simulink model "ForwardKinematic_YuMi"  (R2024a)
(part 14 of 23)

(4872700232219253*sin(q1L))/9007199254740992))/36893488147419103232 - (76229820211215127867025072518845*cos(q2L))/162259276829213363391578010288128 + sin(q2L)*((4872700232219253*cos(q1L))/9007199254740992 + (6283307137322267*sin(q1L))/9007199254740992)))/36893488147419103232))/36893488147419103232))/2451992865385422173373355243440494693789982595493763481600 + (27*cos(q5L)*(((7514214926474921*cos(q4L))/36893488147419103232 + (4503599440548691*sin(q4L))/4503599627370496)*((9007199067919185*cos(q3L)*((56594998190739085871744456992395*cos(q1L))/81129638414606681695789005144064 - (43889380989894851923989405068805*sin(q1L))/81129638414606681695789005144064 + 63594381400292563045725890951477/664613997892457936451903530140172288))/9007199254740992 + (7514214926474921*cos(q3L)*((7514214926474921*cos(q2L)*((6283307137322267*cos(q1L))/9007199254740992 - (4872700232219253*sin(q1L))/9007199254740992))/36893488147419103232 - (76229820211215127867025072518845*cos(q2L))/162259276829213363391578010288128 + sin(q2L)*((4872700232219253*cos(q1L))/9007199254740992 + (6283307137322267*sin(q1L))/9007199254740992)))/36893488147419103232 - sin(q3L)*((76229820211215127867025072518845*sin(q2L))/162259276829213363391578010288128 + cos(q2L)*((4872700232219253*cos(q1L))/9007199254740992 + (6283307137322267*sin(q1L))/9007199254740992) - (7514214926474921*sin(q2L)*((6283307137322267*cos(q1L))/9007199254740992 - (4872700232219253*sin(q1L))/9007199254740992))/36893488147419103232)) - (7514214926474921*sin(q4L)*((9007199067919185*sin(q3L)*((56594998190739085871744456992395*cos(q1L))/81129638414606681695789005144064 - (43889380989894851923989405068805*sin(q1L))/81129638414606681695789005144064 + 63594381400292563045725890951477/664613997892457936451903530140172288))/9007199254740992 + cos(q3L)*((76229820211215127867025072518845*sin(q2L))/162259276829213363391578010288128 + cos(q2L)*((4872700232219253*cos(q1L))/9007199254740992 + (6283307137322267*sin(q1L))/9007199254740992) - (7514214926474921*sin(q2L)*((6283307137322267*cos(q1L))/9007199254740992 - (4872700232219253*sin(q1L))/9007199254740992))/36893488147419103232) + (7514214926474921*sin(q3L)*((7514214926474921*cos(q2L)*((6283307137322267*cos(q1L))/9007199254740992 - (4872700232219253*sin(q1L))/9007199254740992))/36893488147419103232 - (76229820211215127867025072518845*cos(q2L))/162259276829213363391578010288128 + sin(q2L)*((4872700232219253*cos(q1L))/9007199254740992 + (6283307137322267*sin(q1L))/9007199254740992)))/36893488147419103232))/36893488147419103232))/1000 - (202883803014822867*sin(q5L)*(((4503599440548691*cos(q4L))/4503599627370496 - (7514214926474921*sin(q4L))/36893488147419103232)*((9007199067919185*cos(q3L)*((56594998190739085871744456992395*cos(q1L))/81129638414606681695789005144064 - (43889380989894851923989405068805*sin(q1L))/81129638414606681695789005144064 + 63594381400292563045725890951477/664613997892457936451903530140172288))/9007199254740992 + (7514214926474921*cos(q3L)*((7514214926474921*cos(q2L)*((6283307137322267*cos(q1L))/9007199254740992 - (4872700232219253*sin(q1L))/9007199254740992))/36893488147419103232 - (76229820211215127867025072518845*cos(q2L))/162259276829213363391578010288128 + sin(q2L)*((4872700232219253*cos(q1L))/9007199254740992 + (6283307137322267*sin(q1L))/9007199254740992)))/36893488147419103232 - sin(q3L)*((76229820211215127867025072518845*sin(q2L))/162259276829213363391578010288128 + cos(q2L)*((4872700232219253*cos(q1L))/9007199254740992 + (6283307137322267*sin(q1L))/9007199254740992) - (7514214926474921*sin(q2L)*((6283307137322267*cos(q1L))/9007199254740992 - (4872700232219253*sin(q1L))/9007199254740992))/36893488147419103232)) - (7514214926474921*cos(q4L)*((9007199067919185*sin(q3L)*((56594998190739085871744456992395*cos(q1L))/81129638414606681695789005144064 - (43889380989894851923989405068805*sin(q1L))/81129638414606681695789005144064 + 63594381400292563045725890951477/664613997892457936451903530140172288))/9007199254740992 + cos(q3L)*((76229820211215127867025072518845*sin(q2L))/162259276829213363391578010288128 + cos(q2L)*((4872700232219253*cos(q1L))/9007199254740992 + (6283307137322267*sin(q1L))/9007199254740992) - (7514214926474921*sin(q2L)*((6283307137322267*cos(q1L))/9007199254740992 - (4872700232219253*sin(q1L))/9007199254740992))/36893488147419103232) + (7514214926474921*sin(q3L)*((7514214926474921*cos(q2L)*((6283307137322267*cos(q1L))/9007199254740992 - (4872700232219253*sin(q1L))/9007199254740992))/36893488147419103232 - (76229820211215127867025072518845*cos(q2L))/162259276829213363391578010288128 + sin(q2L)*((4872700232219253*cos(q1L))/9007199254740992 + (6283307137322267*sin(q1L))/9007199254740992)))/36893488147419103232))/36893488147419103232))/36893488147419103232000 + (94754841554645069948206780163139*sin(q5L)*(((7514214926474921*cos(q4L))/36893488147419103232 + (4503599440548691*sin(q4L))/4503599627370496)*((9007199067919185*cos(q3L)*((56594998190739085871744456992395*cos(q1L))/81129638414606681695789005144064 - (43889380989894851923989405068805*sin(q1L))/81129638414606681695789005144064 + 63594381400292563045725890951477/664613997892457936451903530140172288))/9007199254740992 + (7514214926474921*cos(q3L)*((7514214926474921*cos(q2L)*((6283307137322267*cos(q1L))/9007199254740992 - (4872700232219253*sin(q1L))/9007199254740992))/36893488147419103232 - (76229820211215127867025072518845*cos(q2L))/162259276829213363391578010288128 + sin(q2L)*((4872700232219253*cos(q1L))/9007199254740992 + (6283307137322267*sin(q1L))/9007199254740992)))/36893488147419103232 - sin(q3L)*((76229820211215127867025072518845*sin(q2L))/162259276829213363391578010288128 + cos(q2L)*((4872700232219253*cos(q1L))/9007199254740992 + (6283307137322267*sin(q1L))/9007199254740992) - (7514214926474921*sin(q2L)*((6283307137322267*cos(q1L))/9007199254740992 - (4872700232219253*sin(q1L))/9007199254740992))/36893488147419103232)) - (7514214926474921*sin(q4L)*((9007199067919185*sin(q3L)*((56594998190739085871744456992395*cos(q1L))/81129638414606681695789005144064 - (43889380989894851923989405068805*sin(q1L))/81129638414606681695789005144064 + 63594381400292563045725890951477/664613997892457936451903530140172288))/9007199254740992 + cos(q3L)*((76229820211215127867025072518845*sin(q2L))/162259276829213363391578010288128 + cos(q2L)*((4872700232219253*cos(q1L))/9007199254740992 + (6283307137322267*sin(q1L))/9007199254740992) - (7514214926474921*sin(q2L)*((6283307137322267*cos(q1L))/9007199254740992 - (4872700232219253*sin(q1L))/9007199254740992))/36893488147419103232) + (7514214926474921*sin(q3L)*((7514214926474921*cos(q2L)*((6283307137322267*cos(q1L))/9007199254740992 - (4872700232219253*sin(q1L))/9007199254740992))/36893488147419103232 - (76229820211215127867025072518845*cos(q2L))/162259276829213363391578010288128 + sin(q2L)*((4872700232219253*cos(q1L))/9007199254740992 + (6283307137322267*sin(q1L))/9007199254740992)))/36893488147419103232))/36893488147419103232))/66461399789245793645190353014017228800, (27*cos(q5L)*(((4503599440548691*cos(q4L))/4503599627370496 - (7514214926474921*sin(q4L))/36893488147419103232)*((9007199067919185*sin(q3L)*((56594998190739085871744456992395*cos(q1L))/81129638414606681695789005144064 - (43889380989894851923989405068805*sin(q1L))/81129638414606681695789005144064 + 63594381400292563045725890951477/664613997892457936451903530140172288))/9007199254740992 + cos(q3L)*((76229820211215127867025072518845*sin(q2L))/162259276829213363391578010288128 + cos(q2L)*((4872700232219253*cos(q1L))/9007199254740992 + (6283307137322267*sin(q1L))/9007199254740992) - (7514214926474921*sin(q2L)*((6283307137322267*cos(q1L))/9007199254740992 - (4872700232219253*sin(q1L))/9007199254740992))/36893488147419103232) + (7514214926474921*sin(q3L)*((7514214926474921*cos(q2L)*((6283307137322267*cos(q1L))/9007199254740992 - (4872700232219253*sin(q1L))/9007199254740992))/36893488147419103232 - (76229820211215127867025072518845*cos(q2L))/162259276829213363391578010288128 + sin(q2L)*((4872700232219253*cos(q1L))/9007199254740992 + (6283307137322267*sin(q1L))/9007199254740992)))/36893488147419103232) + ((234819211581865*cos(q4L))/1152921504606846976 + (9007199067919185*sin(q4L))/9007199254740992)*((425266980168672787164801917791314326747055225795*cos(q1L))/2993155353253689176481146537402947624255349848014848 + (686617165554103949950999710565799465200849541325*cos(q2L))/1461501637330902918203684832716283019655932542976 - (329794241748012540206902858004467560228111939405*sin(q1L))/2993155353253689176481146537402947624255349848014848 - (67682029681889335677290557259385*cos(q2L)*((6283307137322267*cos(q1L))/9007199254740992 - (4872700232219253*sin(q1L))/9007199254740992))/332306998946228968225951765070086144 - (9007199067919185*sin(q2L)*((4872700232219253*cos(q1L))/9007199254740992 + (6283307137322267*sin(q1L))/9007199254740992))/9007199254740992 + 477861849958017465213997854626476001002268408317/24519928653854221733733552434404946937899825954937634816) + (7514214926474921*cos(q4L)*((9007199067919185*cos(q3L)*((56594998190739085871744456992395*cos(q1L))/81129638414606681695789005144064 - (43889380989894851923989405068805*sin(q1L))/81129638414606681695789005144064 + 63594381400292563045725890951477/664613997892457936451903530140172288))/9007199254740992 + (7514214926474921*cos(q3L)*((7514214926474921*cos(q2L)*((6283307137322267*cos(q1L))/9007199254740992 - (4872700232219253*sin(q1L))/9007199254740992))/36893488147419103232 - (76229820211215127867025072518845*cos(q2L))/162259276829213363391578010288128 + sin(q2L)*((4872700232219253*cos(q1L))/9007199254740992 + (6283307137322267*sin(q1L))/9007199254740992)))/36893488147419103232 - sin(q3L)*((76229820211215127867025072518845*sin(q2L))/162259276829213363391578010288128 + cos(q2L)*((4872700232219253*cos(q1L))/9007199254740992 + (6283307137322267*sin(q1L))/9007199254740992) - (7514214926474921*sin(q2L)*((6283307137322267*cos(q1L))/9007199254740992 - (4872700232219253*sin(q1L))/9007199254740992))/36893488147419103232)))/36893488147419103232))/1000 + (94754841554645069948206780163139*sin(q5L)*(((4503599440548691*cos(q4L))/4503599627370496 - (7514214926474921*sin(q4L))/36893488147419103232)*((9007199067919185*sin(q3L)*((56594998190739085871744456992395*cos(q1L))/81129638414606681695789005144064 - (43889380989894851923989405068805*sin(q1L))/81129638414606681695789005144064 + 63594381400292563045725890951477/664613997892457936451903530140172288))/9007199254740992 + cos(q3L)*((76229820211215127867025072518845*sin(q2L))/162259276829213363391578010288128 + cos(q2L)*((4872700232219253*cos(q1L))/9007199254740992 + (6283307137322267*sin(q1L))/9007199254740992) - (7514214926474921*sin(q2L)*((6283307137322267*cos(q1L))/9007199254740992 - (4872700232219253*sin(q1L))/9007199254740992))/36893488147419103232) + (7514214926474921*sin(q3L)*((7514214926474921*cos(q2L)*((6283307137322267*cos(q1L))/9007199254740992 - (4872700232219253*sin(q1L))/9007199254740992))/36893488147419103232 - (76229820211215127867025072518845*cos(q2L))/162259276829213363391578010288128 + sin(q2L)*((4872700232219253*cos(q1L))/9007199254740992 + (6283307137322267*sin(q1L))/9007199254740992)))/36893488147419103232) + ((234819211581865*cos(q4L))/1152921504606846976 + (9007199067919185*sin(q4L))/9007199254740992)*((425266980168672787164801917791314326747055225795*cos(q1L))/2993155353253689176481146537402947624255349848014848 + (686617165554103949950999710565799465200849541325*cos(q2L))/1461501637330902918203684832716283019655932542976 - (329794241748012540206902858004467560228111939405*sin(q1L))/2993155353253689176481146537402947624255349848014848 - (67682029681889335677290557259385*cos(q2L)*((6283307137322267*cos(q1L))/9007199254740992 - (4872700232219253*sin(q1L))/9007199254740992))/332306998946228968225951765070086144 - (9007199067919185*sin(q2L)*((4872700232219253*cos(q1L))/9007199254740992 + (6283307137322267*sin(q1L))/9007199254740992))/9007199254740992 + 477861849958017465213997854626476001002268408317/24519928653854221733733552434404946937899825954937634816) + (7514214926474921*cos(q4L)*((9007199067919185*cos(q3L)*((56594998190739085871744456992395*cos(q1L))/81129638414606681695789005144064 - (43889380989894851923989405068805*sin(q1L))/81129638414606681695789005144064 + 63594381400292563045725890951477/664613997892457936451903530140172288))/9007199254740992 + (7514214926474921*cos(q3L)*((7514214926474921*cos(q2L)*((6283307137322267*cos(q1L))/9007199254740992 - (4872700232219253*sin(q1L))/9007199254740992))/36893488147419103232 - (76229820211215127867025072518845*cos(q2L))/162259276829213363391578010288128 + sin(q2L)*((4872700232219253*cos(q1L))/9007199254740992 + (6283307137322267*sin(q1L))/9007199254740992)))/36893488147419103232 - sin(q3L)*((76229820211215127867025072518845*sin(q2L))/162259276829213363391578010288128 + cos(q2L)*((4872700232219253*cos(q1L))/9007199254740992 + (6283307137322267*sin(q1L))/9007199254740992) - (7514214926474921*sin(q2L)*((6283307137322267*cos(q1L))/9007199254740992 - (4872700232219253*sin(q1L))/9007199254740992))/36893488147419103232)))/36893488147419103232))/66461399789245793645190353014017228800 - (712008244765680093343103025701132101054572137019*cos(q5L)*(((7514214926474921*cos(q4L))/36893488147419103232 + (4503599440548691*sin(q4L))/4503599627370496)*((9007199067919185*sin(q3L)*((56594998190739085871744456992395*cos(q1L))/81129638414606681695789005144064 - (43889380989894851923989405068805*sin(q1L))/81129638414606681695789005144064 + 63594381400292563045725890951477/664613997892457936451903530140172288))/9007199254740992 + cos(q3L)*((76229820211215127867025072518845*sin(q2L))/162259276829213363391578010288128 + cos(q2L)*((4872700232219253*cos(q1L))/9007199254740992 + (6283307137322267*sin(q1L))/9007199254740992) - (7514214926474921*sin(q2L)*((6283307137322267*cos(q1L))/9007199254740992 - (4872700232219253*sin(q1L))/9007199254740992))/36893488147419103232) + (7514214926474921*sin(q3L)*((7514214926474921*cos(q2L)*((6283307137322267*cos(q1L))/9007199254740992 - (4872700232219253*sin(q1L))/9007199254740992))/36893488147419103232 - (76229820211215127867025072518845*cos(q2L))/162259276829213363391578010288128 + sin(q2L)*((4872700232219253*cos(q1L))/9007199254740992 + (6283307137322267*sin(q1L))/9007199254740992)))/36893488147419103232) - ((9007199067919185*cos(q4L))/9007199254740992 - (234819211581865*sin(q4L))/1152921504606846976)*((425266980168672787164801917791314326747055225795*cos(q1L))/2993155353253689176481146537402947624255349848014848 + (686617165554103949950999710565799465200849541325*cos(q2L))/1461501637330902918203684832716283019655932542976 - (329794241748012540206902858004467560228111939405*sin(q1L))/2993155353253689176481146537402947624255349848014848 - (67682029681889335677290557259385*cos(q2L)*((6283307137322267*cos(q1L))/9007199254740992 - (4872700232219253*sin(q1L))/9007199254740992))/332306998946228968225951765070086144 - (9007199067919185*sin(q2L)*((4872700232219253*cos(q1L))/9007199254740992 + (6283307137322267*sin(q1L))/9007199254740992))/9007199254740992 + 477861849958017465213997854626476001002268408317/24519928653854221733733552434404946937899825954937634816) + (7514214926474921*sin(q4L)*((9007199067919185*cos(q3L)*((56594998190739085871744456992395*cos(q1L))/81129638414606681695789005144064 - (43889380989894851923989405068805*sin(q1L))/81129638414606681695789005144064 + 63594381400292563045725890951477/664613997892457936451903530140172288))/9007199254740992 + (7514214926474921*cos(q3L)*((7514214926474921*cos(q2L)*((6283307137322267*cos(q1L))/9007199254740992 - (4872700232219253*sin(q1L))/9007199254740992))/36893488147419103232 - (76229820211215127867025072518845*cos(q2L))/162259276829213363391578010288128 + sin(q2L)*((4872700232219253*cos(q1L))/9007199254740992 + (6283307137322267*sin(q1L))/9007199254740992)))/36893488147419103232 - sin(q3L)*((76229820211215127867025072518845*sin(q2L))/162259276829213363391578010288128 + cos(q2L)*((4872700232219253*cos(q1L))/9007199254740992 + (6283307137322267*sin(q1L))/9007199254740992) - (7514214926474921*sin(q2L)*((6283307137322267*cos(q1L))/9007199254740992 - (4872700232219253*sin(q1L))/9007199254740992))/36893488147419103232)))/36893488147419103232))/2451992865385422173373355243440494693789982595493763481600 - (81*((4503599440548691*cos(q4L))/4503599627370496 - (7514214926474921*sin(q4L))/36893488147419103232)*((9007199067919185*sin(q3L)*((56594998190739085871744456992395*cos(q1L))/81129638414606681695789005144064 - (43889380989894851923989405068805*sin(q1L))/81129638414606681695789005144064 + 63594381400292563045725890951477/664613997892457936451903530140172288))/9007199254740992 + cos(q3L)*((76229820211215127867025072518845*sin(q2L))/162259276829213363391578010288128 + cos(q2L)*((4872700232219253*cos(q1L))/9007199254740992 + (6283307137322267*sin(q1L))/9007199254740992) - (7514214926474921*sin(q2L)*((6283307137322267*cos(q1L))/9007199254740992 - (4872700232219253*sin(q1L))/9007199254740992))/36893488147419103232) + (7514214926474921*sin(q3L)*((7514214926474921*cos(q2L)*((6283307137322267*cos(q1L))/9007199254740992 - (4872700232219253*sin(q1L))/9007199254740992))/36893488147419103232 - (76229820211215127867025072518845*cos(q2L))/162259276829213363391578010288128 + sin(q2L)*((4872700232219253*cos(q1L))/9007199254740992 + (6283307137322267*sin(q1L))/9007199254740992)))/36893488147419103232))/2000 + (81222263116692158804177042061221826384594597321566869716687*((7514214926474921*cos(q4L))/36893488147419103232 + (4503599440548691*sin(q4L))/4503599627370496)*((9007199067919185*sin(q3L)*((56594998190739085871744456992395*cos(q1L))/81129638414606681695789005144064 - (43889380989894851923989405068805*sin(q1L))/81129638414606681695789005144064 + 63594381400292563045725890951477/664613997892457936451903530140172288))/9007199254740992 + cos(q3L)*((76229820211215127867025072518845*sin(q2L))/162259276829213363391578010288128 + cos(q2L)*((4872700232219253*cos(q1L))/9007199254740992 + (6283307137322267*sin(q1L))/9007199254740992) - (7514214926474921*sin(q2L)*((6283307137322267*cos(q1L))/9007199254740992 - (4872700232219253*sin(q1L))/9007199254740992))/36893488147419103232) + (7514214926474921*sin(q3L)*((7514214926474921*cos(q2L)*((6283307137322267*cos(q1L))/9007199254740992 - (4872700232219253*sin(q1L))/9007199254740992))/36893488147419103232 - (76229820211215127867025072518845*cos(q2L))/162259276829213363391578010288128 + sin(q2L)*((4872700232219253*cos(q1L))/9007199254740992 + (6283307137322267*sin(q1L))/9007199254740992)))/36893488147419103232))/306499108173177771671669405430061836723747824436720435200000 + (202883803014822867*sin(q5L)*(((7514214926474921*cos(q4L))/36893488147419103232 + (4503599440548691*sin(q4L))/4503599627370496)*((9007199067919185*sin(q3L)*((56594998190739085871744456992395*cos(q1L))/81129638414606681695789005144064 - (43889380989894851923989405068805*sin(q1L))/81129638414606681695789005144064 + 63594381400292563045725890951477/664613997892457936451903530140172288))/9007199254740992 + cos(q3L)*((76229820211215127867025072518845*sin(q2L))/162259276829213363391578010288128 + cos(q2L)*((4872700232219253*cos(q1L))/9007199254740992 + (6283307137322267*sin(q1L))/9007199254740992) - (7514214926474921*sin(q2L)*((6283307137322267*cos(q1L))/9007199254740992 - (4872700232219253*sin(q1L))/9007199254740992))/36893488147419103232) + (7514214926474921*sin(q3L)*((7514214926474921*cos(q2L)*((6283307137322267*cos(q1L))/9007199254740992 - (4872700232219253*sin(q1L))/9007199254740992))/36893488147419103232 - (76229820211215127867025072518845*cos(q2L))/162259276829213363391578010288128 + sin(q2L)*((4872700232219253*cos(q1L))/9007199254740992 + (6283307137322267*sin(q1L))/9007199254740992)))/36893488147419103232) - ((9007199067919185*cos(q4L))/9007199254740992 - (234819211581865*sin(q4L))/1152921504606846976)*((425266980168672787164801917791314326747055225795*cos(q1L))/2993155353253689176481146537402947624255349848014848 + (686617165554103949950999710565799465200849541325*cos(q2L))/1461501637330902918203684832716283019655932542976 - (329794241748012540206902858004467560228111939405*sin(q1L))/2993155353253689176481146537402947624255349848014848 - (67682029681889335677290557259385*cos(q2L)*((6283307137322267*cos(q1L))/9007199254740992 - (4872700232219253*sin(q1L))/9007199254740992))/332306998946228968225951765070086144 - (9007199067919185*sin(q2L)*((4872700232219253*cos(q1L))/9007199254740992 + (6283307137322267*sin(q1L))/9007199254740992))/9007199254740992 + 477861849958017465213997854626476001002268408317/24519928653854221733733552434404946937899825954937634816) + (7514214926474921*sin(q4L)*((9007199067919185*cos(q3L)*((56594998190739085871744456992395*cos(q1L))/81129638414606681695789005144064 - (43889380989894851923989405068805*sin(q1L))/81129638414606681695789005144064 + 63594381400292563045725890951477/664613997892457936451903530140172288))/9007199254740992 + (7514214926474921*cos(q3L)*((7514214926474921*cos(q2L)*((6283307137322267*cos(q1L))/9007199254740992 - (4872700232219253*sin(q1L))/9007199254740992))/36893488147419103232 - (76229820211215127867025072518845*cos(q2L))/162259276829213363391578010288128 + sin(q2L)*((4872700232219253*cos(q1L))/9007199254740992 + (6283307137322267*sin(q1L))/9007199254740992)))/36893488147419103232 - sin(q3L)*((76229820211215127867025072518845*sin(q2L))/162259276829213363391578010288128 + cos(q2L)*((4872700232219253*cos(q1L))/9007199254740992 + (6283307137322267*sin(q1L))/9007199254740992) - (7514214926474921*sin(q2L)*((6283307137322267*cos(q1L))/9007199254740992 - (4872700232219253*sin(q1L))/9007199254740992))/36893488147419103232)))/36893488147419103232))/36893488147419103232000 - (81222263116692158804177042061221826384594597321566869716687*((9007199067919185*cos(q4L))/9007199254740992 - (234819211581865*sin(q4L))/1152921504606846976)*((425266980168672787164801917791314326747055225795*cos(q1L))/2993155353253689176481146537402947624255349848014848 + (686617165554103949950999710565799465200849541325*cos(q2L))/1461501637330902918203684832716283019655932542976 - (329794241748012540206902858004467560228111939405*sin(q1L))/2993155353253689176481146537402947624255349848014848 - (67682029681889335677290557259385*cos(q2L)*((6283307137322267*cos(q1L))/9007199254740992 - (4872700232219253*sin(q1L))/9007199254740992))/332306998946228968225951765070086144 - (9007199067919185*sin(q2L)*((4872700232219253*cos(q1L))/9007199254740992 + (6283307137322267*sin(q1L))/9007199254740992))/9007199254740992 + 477861849958017465213997854626476001002268408317/24519928653854221733733552434404946937899825954937634816))/306499108173177771671669405430061836723747824436720435200000 - (81*((234819211581865*cos(q4L))/1152921504606846976 + (9007199067919185*sin(q4L))/9007199254740992)*((425266980168672787164801917791314326747055225795*cos(q1L))/2993155353253689176481146537402947624255349848014848 + (686617165554103949950999710565799465200849541325*cos(q2L))/1461501637330902918203684832716283019655932542976 - (329794241748012540206902858004467560228111939405*sin(q1L))/2993155353253689176481146537402947624255349848014848 - (67682029681889335677290557259385*cos(q2L)*((6283307137322267*cos(q1L))/9007199254740992 - (4872700232219253*sin(q1L))/9007199254740992))/332306998946228968225951765070086144 - (9007199067919185*sin(q2L)*((4872700232219253*cos(q1L))/9007199254740992 + (6283307137322267*sin(q1L))/9007199254740992))/9007199254740992 + 477861849958017465213997854626476001002268408317/24519928653854221733733552434404946937899825954937634816))/2000 - (27*cos(q6L)*(cos(q5L)*(((4503599440548691*cos(q4L))/4503599627370496 - (7514214926474921*sin(q4L))/36893488147419103232)*((9007199067919185*sin(q3L)*((56594998190739085871744456992395*cos(q1L))/81129638414606681695789005144064 - (43889380989894851923989405068805*sin(q1L))/81129638414606681695789005144064 + 63594381400292563045725890951477/664613997892457936451903530140172288))/9007199254740992 + cos(q3L)*((76229820211215127867025072518845*sin(q2L))/162259276829213363391578010288128 + cos(q2L)*((4872700232219253*cos(q1L))/9007199254740992 + (6283307137322267*sin(q1L))/9007199254740992) - (7514214926474921*sin(q2L)*((6283307137322267*cos(q1L))/9007199254740992 - (4872700232219253*sin(q1L))/9007199254740992))/36893488147419103232) + (7514214926474921*sin(q3L)*((7514214926474921*cos(q2L)*((6283307137322267*cos(q1L))/9007199254740992 - (4872700232219253*sin(q1L))/9007199254740992))/36893488147419103232 - (76229820211215127867025072518845*cos(q2L))/162259276829213363391578010288128 + sin(q2L)*((4872700232219253*cos(q1L))/9007199254740992 + (6283307137322267*sin(q1L))/9007199254740992)))/36893488147419103232) + ((234819211581865*cos(q4L))/1152921504606846976 + (9007199067919185*sin(q4L))/9007199254740992)*((425266980168672787164801917791314326747055225795*cos(q1L))/2993155353253689176481146537402947624255349848014848 + (686617165554103949950999710565799465200849541325*cos(q2L))/1461501637330902918203684832716283019655932542976 - (329794241748012540206902858004467560228111939405*sin(q1L))/2993155353253689176481146537402947624255349848014848 - (67682029681889335677290557259385*cos(q2L)*((6283307137322267*cos(q1L))/9007199254740992 - (4872700232219253*sin(q1L))/9007199254740992))/332306998946228968225951765070086144 - (9007199067919185*sin(q2L)*((4872700232219253*cos(q1L))/9007199254740992 + (6283307137322267*sin(q1L))/9007199254740992))/9007199254740992 + 477861849958017465213997854626476001002268408317/24519928653854221733733552434404946937899825954937634816) + (7514214926474921*cos(q4L)*((9007199067919185*cos(q3L)*((56594998190739085871744456992395*cos(q1L))/81129638414606681695789005144064 - (43889380989894851923989405068805*sin(q1L))/81129638414606681695789005144064 + 63594381400292563045725890951477/664613997892457936451903530140172288))/9007199254740992 + (7514214926474921*cos(q3L)*((7514214926474921*cos(q2L)*((6283307137322267*cos(q1L))/9007199254740992 - (4872700232219253*sin(q1L))/9007199254740992))/36893488147419103232 - (76229820211215127867025072518845*cos(q2L))/162259276829213363391578010288128 + sin(q2L)*((4872700232219253*cos(q1L))/9007199254740992 + (6283307137322267*sin(q1L))/9007199254740992)))/36893488147419103232 - sin(q3L)*((76229820211215127867025072518845*sin(q2L))/162259276829213363391578010288128 + cos(q2L)*((4872700232219253*cos(q1L))/9007199254740992 + (6283307137322267*sin(q1L))/9007199254740992) - (7514214926474921*sin(q2L)*((6283307137322267*cos(q1L))/9007199254740992 - (4872700232219253*sin(q1L))/9007199254740992))/36893488147419103232)))/36893488147419103232) + (7514214926474921*sin(q5L)*(((7514214926474921*cos(q4L))/36893488147419103232 + (4503599440548691*sin(q4L))/4503599627370496)*((9007199067919185*sin(q3L)*((56594998190739085871744456992395*cos(q1L))/81129638414606681695789005144064 - (43889380989894851923989405068805*sin(q1L))/81129638414606681695789005144064 + 63594381400292563045725890951477/664613997892457936451903530140172288))/9007199254740992 + cos(q3L)*((76229820211215127867025072518845*sin(q2L))/162259276829213363391578010288128 + cos(q2L)*((4872700232219253*cos(q1L))/9007199254740992 + (6283307137322267*sin(q1L))/9007199254740992) - (7514214926474921*sin(q2L)*((6283307137322267*cos(q1L))/9007199254740992 - (4872700232219253*sin(q1L))/9007199254740992))/36893488147419103232) + (7514214926474921*sin(q3L)*((7514214926474921*cos(q2L)*((6283307137322267*cos(q1L))/9007199254740992 - (4872700232219253*sin(q1L))/9007199254740992))/36893488147419103232 - (76229820211215127867025072518845*cos(q2L))/162259276829213363391578010288128 + sin(q2L)*((4872700232219253*cos(q1L))/9007199254740992 + (6283307137322267*sin(q1L))/9007199254740992)))/36893488147419103232) - ((9007199067919185*cos(q4L))/9007199254740992 - (234819211581865*sin(q4L))/1152921504606846976)*((425266980168672787164801917791314326747055225795*cos(q1L))/2993155353253689176481146537402947624255349848014848 + (686617165554103949950999710565799465200849541325*cos(q2L))/1461501637330902918203684832716283019655932542976 - (329794241748012540206902858004467560228111939405*sin(q1L))/2993155353253689176481146537402947624255349848014848 - (67682029681889335677290557259385*cos(q2L)*((6283307137322267*cos(q1L))/9007199254740992 - (4872700232219253*sin(q1L))/9007199254740992))/332306998946228968225951765070086144 - (9007199067919185*sin(q2L)*((4872700232219253*cos(q1L))/9007199254740992 + (6283307137322267*sin(q1L))/9007199254740992))/9007199254740992 + 477861849958017465213997854626476001002268408317/24519928653854221733733552434404946937899825954937634816) + (7514214926474921*sin(q4L)*((9007199067919185*cos(q3L)*((56594998190739085871744456992395*cos(q1L))/81129638414606681695789005144064 - (43889380989894851923989405068805*sin(q1L))/81129638414606681695789005144064 + 63594381400292563045725890951477/664613997892457936451903530140172288))/9007199254740992 + (7514214926474921*cos(q3L)*((7514214926474921*cos(q2L)*((6283307137322267*cos(q1L))/9007199254740992 - (4872700232219253*sin(q1L))/9007199254740992))/36893488147419103232 - (76229820211215127867025072518845*cos(q2L))/162259276829213363391578010288128 + sin(q2L)*((4872700232219253*cos(q1L))/9007199254740992 + (6283307137322267*sin(q1L))/9007199254740992)))/36893488147419103232 - sin(q3L)*((76229820211215127867025072518845*sin(q2L))/162259276829213363391578010288128 + cos(q2L)*((4872700232219253*cos(q1L))/9007199254740992 + (6283307137322267*sin(q1L))/9007199254740992) - (7514214926474921*sin(q2L)*((6283307137322267*cos(q1L))/9007199254740992 - (4872700232219253*sin(q1L))/9007199254740992))/36893488147419103232)))/36893488147419103232))/36893488147419103232))/1000 - (2436553109258773196144549622003023*cos(q6L)*(sin(q5L)*(((4503599440548691*cos(q4L))/4503599627370496 - (7514214926474921*sin(q4L))/36893488147419103232)*((9007199067919185*sin(q3L)*((56594998190739085871744456992395*cos(q1L))/81129638414606681695789005144064 - (43889380989894851923989405068805*sin(q1L))/81129638414606681695789005144064 + 63594381400292563045725890951477/664613997892457936451903530140172288))/9007199254740992 + cos(q3L)*((76229820211215127867025072518845*sin(q2L))/162259276829213363391578010288128 + cos(q2L)*((4872700232219253*cos(q1L))/9007199254740992 + (6283307137322267*sin(q1L))/9007199254740992) - (7514214926474921*sin(q2L)*((6283307137322267*cos(q1L))/9007199254740992 - (4872700232219253*sin(q1L))/9007199254740992))/36893488147419103232) + (7514214926474921*sin(q3L)*((7514214926474921*cos(q2L)*((6283307137322267*cos(q1L))/9007199254740992 - (4872700232219253*sin(q1L))/9007199254740992))/36893488147419103232 - (76229820211215127867025072518845*cos(q2L))/162259276829213363391578010288128 + sin(q2L)*((4872700232219253*cos(q1L))/9007199254740992 + (6283307137322267*sin(q1L))/9007199254740992)))/36893488147419103232) + ((234819211581865*cos(q4L))/1152921504606846976 + (9007199067919185*sin(q4L))/9007199254740992)*((425266980168672787164801917791314326747055225795*cos(q1L))/2993155353253689176481146537402947624255349848014848 + (686617165554103949950999710565799465200849541325*cos(q2L))/1461501637330902918203684832716283019655932542976 - (329794241748012540206902858004467560228111939405*sin(q1L))/2993155353253689176481146537402947624255349848014848 - (67682029681889335677290557259385*cos(q2L)*((6283307137322267*cos(q1L))/9007199254740992 - (4872700232219253*sin(q1L))/9007199254740992))/332306998946228968225951765070086144 - (9007199067919185*sin(q2L)*((4872700232219253*cos(q1L))/9007199254740992 + (6283307137322267*sin(q1L))/9007199254740992))/9007199254740992 + 477861849958017465213997854626476001002268408317/24519928653854221733733552434404946937899825954937634816) + (7514214926474921*cos(q4L)*((9007199067919185*cos(q3L)*((56594998190739085871744456992395*cos(q1L))/81129638414606681695789005144064 - (43889380989894851923989405068805*sin(q1L))/81129638414606681695789005144064 + 63594381400292563045725890951477/664613997892457936451903530140172288))/9007199254740992 + (7514214926474921*cos(q3L)*((7514214926474921*cos(q2L)*((6283307137322267*cos(q1L))/9007199254740992 - (4872700232219253*sin(q1L))/9007199254740992))/36893488147419103232 - (76229820211215127867025072518845*cos(q2L))/162259276829213363391578010288128 + sin(q2L)*((4872700232219253*cos(q1L))/9007199254740992 + (6283307137322267*sin(q1L))/9007199254740992)))/36893488147419103232 - sin(q3L)*((76229820211215127867025072518845*sin(q2L))/162259276829213363391578010288128 + cos(q2L)*((4872700232219253*cos(q1L))/9007199254740992 + (6283307137322267*sin(q1L))/9007199254740992) - (7514214926474921*sin(q2L)*((6283307137322267*cos(q1L))/9007199254740992 - (4872700232219253*sin(q1L))/9007199254740992))/36893488147419103232)))/36893488147419103232) - (7514214926474921*cos(q5L)*(((7514214926474921*cos(q4L))/36893488147419103232 + (4503599440548691*sin(q4L))/4503599627370496)*((9007199067919185*sin(q3L)*((56594998190739085871744456992395*cos(q1L))/81129638414606681695789005144064 - (43889380989894851923989405068805*sin(q1L))/81129638414606681695789005144064 + 63594381400292563045725890951477/664613997892457936451903530140172288))/9007199254740992 + cos(q3L)*((76229820211215127867025072518845*sin(q2L))/162259276829213363391578010288128 + cos(q2L)*((4872700232219253*cos(q1L))/9007199254740992 + (6283307137322267*sin(q1L))/9007199254740992) - (7514214926474921*sin(q2L)*((6283307137322267*cos(q1L))/9007199254740992 - (4872700232219253*sin(q1L))/9007199254740992))/36893488147419103232) + (7514214926474921*sin(q3L)*((7514214926474921*cos(q2L)*((6283307137322267*cos(q1L))/9007199254740992 - (4872700232219253*sin(q1L))/9007199254740992))/36893488147419103232 - (76229820211215127867025072518845*cos(q2L))/162259276829213363391578010288128 + sin(q2L)*((4872700232219253*cos(q1L))/9007199254740992 + (6283307137322267*sin(q1L))/9007199254740992)))/36893488147419103232) - ((9007199067919185*cos(q4L))/9007199254740992 - (234819211581865*sin(q4L))/1152921504606846976)*((425266980168672787164801917791314326747055225795*cos(q1L))/2993155353253689176481146537402947624255349848014848 + (686617165554103949950999710565799465200849541325*cos(q2L))/1461501637330902918203684832716283019655932542976 - (329794241748012540206902858004467560228111939405*sin(q1L))/2993155353253689176481146537402947624255349848014848 - (67682029681889335677290557259385*cos(q2L)*((6283307137322267*cos(q1L))/9007199254740992 - (4872700232219253*sin(q1L))/9007199254740992))/332306998946228968225951765070086144 - (9007199067919185*sin(q2L)*((4872700232219253*cos(q1L))/9007199254740992 + (6283307137322267*sin(q1L))/9007199254740992))/9007199254740992 + 477861849958017465213997854626476001002268408317/24519928653854221733733552434404946937899825954937634816) + (7514214926474921*sin(q4L)*((9007199067919185*cos(q3L)*((56594998190739085871744456992395*cos(q1L))/81129638414606681695789005144064 - (43889380989894851923989405068805*sin(q1L))/81129638414606681695789005144064 + 63594381400292563045725890951477/664613997892457936451903530140172288))/9007199254740992 + (7514214926474921*cos(q3L)*((7514214926474921*cos(q2L)*((6283307137322267*cos(q1L))/9007199254740992 - (4872700232219253*sin(q1L))/9007199254740992))/36893488147419103232 - (76229820211215127867025072518845*cos(q2L))/162259276829213363391578010288128 + sin(q2L)*((4872700232219253*cos(q1L))/9007199254740992 + (6283307137322267*sin(q1L))/9007199254740992)))/36893488147419103232 - sin(q3L)*((76229820211215127867025072518845*sin(q2L))/162259276829213363391578010288128 + cos(q2L)*((4872700232219253*cos(q1L))/9007199254740992 + (6283307137322267*sin(q1L))/9007199254740992) - (7514214926474921*sin(q2L)*((6283307137322267*cos(q1L))/9007199254740992 - (4872700232219253*sin(q1L))/9007199254740992))/36893488147419103232)))/36893488147419103232))/36893488147419103232))/332306998946228968225951765070086144000 + (324259171862923063*sin(q6L)*(cos(q5L)*(((4503599440548691*cos(q4L))/4503599627370496 - (7514214926474921*sin(q4L))/36893488147419103232)*((9007199067919185*sin(q3L)*((56594998190739085871744456992395*cos(q1L))/81129638414606681695789005144064 - (43889380989894851923989405068805*sin(q1L))/81129638414606681695789005144064 + 63594381400292563045725890951477/664613997892457936451903530140172288))/9007199254740992 + cos(q3L)*((76229820211215127867025072518845*sin(q2L))/162259276829213363391578010288128 + cos(q2L)*((4872700232219253*cos(q1L))/9007199254740992 + (6283307137322267*sin(q1L))/9007199254740992) - (7514214926474921*sin(q2L)*((6283307137322267*cos(q1L))/9007199254740992 - (4872700232219253*sin(q1L))/9007199254740992))/36893488147419103232) + (7514214926474921*sin(q3L)*((7514214926474921*cos(q2L)*((6283307137322267*cos(q1L))/9007199254740992 - (4872700232219253*sin(q1L))/9007199254740992))/36893488147419103232 - (76229820211215127867025072518845*cos(q2L))/162259276829213363391578010288128 + sin(q2L)*((4872700232219253*cos(q1L))/9007199254740992 + (6283307137322267*sin(q1L))/9007199254740992)))/36893488147419103232) + ((234819211581865*cos(q4L))/1152921504606846976 + (9007199067919185*sin(q4L))/9007199254740992)*((425266980168672787164801917791314326747055225795*cos(q1L))/2993155353253689176481146537402947624255349848014848 + (686617165554103949950999710565799465200849541325*cos(q2L))/1461501637330902918203684832716283019655932542976 - (329794241748012540206902858004467560228111939405*sin(q1L))/2993155353253689176481146537402947624255349848014848 - (67682029681889335677290557259385*cos(q2L)*((6283307137322267*cos(q1L))/9007199254740992 - (4872700232219253*sin(q1L))/9007199254740992))/332306998946228968225951765070086144 - (9007199067919185*sin(q2L)*((4872700232219253*cos(q1L))/9007199254740992 + (6283307137322267*sin(q1L))/9007199254740992))/9007199254740992 + 477861849958017465213997854626476001002268408317/24519928653854221733733552434404946937899825954937634816) + (7514214926474921*cos(q4L)*((9007199067919185*cos(q3L)*((56594998190739085871744456992395*cos(q1L))/81129638414606681695789005144064 - (43889380989894851923989405068805*sin(q1L))/81129638414606681695789005144064 + 63594381400292563045725890951477/664613997892457936451903530140172288))/9007199254740992 + (7514214926474921*cos(q3L)*((7514214926474921*cos(q2L)*((6283307137322267*cos(q1L))/9007199254740992 - (4872700232219253*sin(q1L))/9007199254740992))/36893488147419103232 - (76229820211215127867025072518845*cos(q2L))/162259276829213363391578010288128 + sin(q2L)*((4872700232219253*cos(q1L))/9007199254740992 + (6283307137322267*sin(q1L))/9007199254740992)))/36893488147419103232 - sin(q3L)*((76229820211215127867025072518845*sin(q2L))/162259276829213363391578010288128 + cos(q2L)*((4872700232219253*cos(q1L))/9007199254740992 + (6283307137322267*sin(q1L))/9007199254740992) - (7514214926474921*sin(q2L)*((6283307137322267*cos(q1L))/9007199254740992 - (4872700232219253*sin(q1L))/9007199254740992))/36893488147419103232)))/36893488147419103232) + (7514214926474921*sin(q5L)*(((7514214926474921*cos(q4L))/36893488147419103232 + (4503599440548691*sin(q4L))/4503599627370496)*((9007199067919185*sin(q3L)*((56594998190739085871744456992395*cos(q1L))/81129638414606681695789005144064 - (43889380989894851923989405068805*sin(q1L))/81129638414606681695789005144064 + 63594381400292563045725890951477/664613997892457936451903530140172288))/9007199254740992 + cos(q3L)*((76229820211215127867025072518845*sin(q2L))/162259276829213363391578010288128 + cos(q2L)*((4872700232219253*cos(q1L))/9007199254740992 + (6283307137322267*sin(q1L))/9007199254740992) - (7514214926474921*sin(q2L)*((6283307137322267*cos(q1L))/9007199254740992 - (4872700232219253*sin(q1L))/9007199254740992))/36893488147419103232) + (7514214926474921*sin(q3L)*((7514214926474921*cos(q2L)*((6283307137322267*cos(q1L))/9007199254740992 - (4872700232219253*sin(q1L))/9007199254740992))/36893488147419103232 - (76229820211215127867025072518845*cos(q2L))/162259276829213363391578010288128 + sin(q2L)*((4872700232219253*cos(q1L))/9007199254740992 + (6283307137322267*sin(q1L))/9007199254740992)))/36893488147419103232) - ((9007199067919185*cos(q4L))/9007199254740992 - (234819211581865*sin(q4L))/1152921504606846976)*((425266980168672787164801917791314326747055225795*cos(q1L))/2993155353253689176481146537402947624255349848014848 + (686617165554103949950999710565799465200849541325*cos(q2L))/1461501637330902918203684832716283019655932542976 - (329794241748012540206902858004467560228111939405*sin(q1L))/2993155353253689176481146537402947624255349848014848 - (67682029681889335677290557259385*cos(q2L)*((6283307137322267*cos(q1L))/9007199254740992 - (4872700232219253*sin(q1L))/9007199254740992))/332306998946228968225951765070086144 - (9007199067919185*sin(q2L)*((4872700232219253*cos(q1L))/9007199254740992 + (6283307137322267*sin(q1L))/9007199254740992))/9007199254740992 + 477861849958017465213997854626476001002268408317/24519928653854221733733552434404946937899825954937634816) + (7514214926474921*sin(q4L)*((9007199067919185*cos(q3L)*((56594998190739085871744456992395*cos(q1L))/81129638414606681695789005144064 - (43889380989894851923989405068805*sin(q1L))/81129638414606681695789005144064 + 63594381400292563045725890951477/664613997892457936451903530140172288))/9007199254740992 + (7514214926474921*cos(q3L)*((7514214926474921*cos(q2L)*((6283307137322267*cos(q1L))/9007199254740992 - (4872700232219253*sin(q1L))/9007199254740992))/36893488147419103232 - (76229820211215127867025072518845*cos(q2L))/162259276829213363391578010288128 + sin(q2L)*((4872700232219253*cos(q1L))/9007199254740992 + (6283307137322267*sin(q1L))/9007199254740992)))/36893488147419103232 - sin(q3L)*((76229820211215127867025072518845*sin(q2L))/162259276829213363391578010288128 + cos(q2L)*((4872700232219253*cos(q1L))/9007199254740992 + (6283307137322267*sin(q1L))/9007199254740992) - (7514214926474921*sin(q2L)*((6283307137322267*cos(q1L))/9007199254740992 - (4872700232219253*sin(q1L))/9007199254740992))/36893488147419103232)))/36893488147419103232))/36893488147419103232))/9007199254740992000 - (202883803014822867*sin(q6L)*(sin(q5L)*(((4503599440548691*cos(q4L))/4503599627370496 - (7514214926474921*sin(q4L))/36893488147419103232)*((9007199067919185*sin(q3L)*((56594998190739085871744456992395*cos(q1L))/81129638414606681695789005144064 - (43889380989894851923989405068805*sin(q1L))/81129638414606681695789005144064 + 63594381400292563045725890951477/664613997892457936451903530140172288))/9007199254740992 + cos(q3L)*((76229820211215127867025072518845*sin(q2L))/162259276829213363391578010288128 + cos(q2L)*((4872700232219253*cos(q1L))/9007199254740992 + (6283307137322267*sin(q1L))/9007199254740992) - (7514214926474921*sin(q2L)*((6283307137322267*cos(q1L))/9007199254740992 - (4872700232219253*sin(q1L))/9007199254740992))/36893488147419103232) + (7514214926474921*sin(q3L)*((7514214926474921*cos(q2L)*((6283307137322267*cos(q1L))/9007199254740992 - (4872700232219253*sin(q1L))/9007199254740992))/36893488147419103232 - (76229820211215127867025072518845*cos(q2L))/162259276829213363391578010288128 + sin(q2L)*((4872700232219253*cos(q1L))/9007199254740992 + (6283307137322267*sin(q1L))/9007199254740992)))/36893488147419103232) + ((234819211581865*cos(q4L))/1152921504606846976 + (9007199067919185*sin(q4L))/9007199254740992)*((425266980168672787164801917791314326747055225795*cos(q1L))/2993155353253689176481146537402947624255349848014848 + (686617165554103949950999710565799465200849541325*cos(q2L))/1461501637330902918203684832716283019655932542976 - (329794241748012540206902858004467560228111939405*sin(q1L))/2993155353253689176481146537402947624255349848014848 - (67682029681889335677290557259385*cos(q2L)*((6283307137322267*cos(q1L))/9007199254740992 - (4872700232219253*sin(q1L))/9007199254740992))/332306998946228968225951765070086144 - (9007199067919185*sin(q2L)*((4872700232219253*cos(q1L))/9007199254740992 + (6283307137322267*sin(q1L))/9007199254740992))/9007199254740992 + 477861849958017465213997854626476001002268408317/24519928653854221733733552434404946937899825954937634816) + (7514214926474921*cos(q4L)*((9007199067919185*cos(q3L)*((56594998190739085871744456992395*cos(q1L))/81129638414606681695789005144064 - (43889380989894851923989405068805*sin(q1L))/81129638414606681695789005144064 + 63594381400292563045725890951477/664613997892457936451903530140172288))/9007199254740992 + (7514214926474921*cos(q3L)*((7514214926474921*cos(q2L)*((6283307137322267*cos(q1L))/9007199254740992 - (4872700232219253*sin(q1L))/9007199254740992))/36893488147419103232 - (76229820211215127867025072518845*cos(q2L))/162259276829213363391578010288128 + sin(q2L)*((4872700232219253*cos(q1L))/9007199254740992 + (6283307137322267*sin(q1L))/9007199254740992)))/36893488147419103232 - sin(q3L)*((76229820211215127867025072518845*sin(q2L))/162259276829213363391578010288128 + cos(q2L)*((4872700232219253*cos(q1L))/9007199254740992 + (6283307137322267*sin(q1L))/9007199254740992) - (7514214926474921*sin(q2L)*((6283307137322267*cos(q1L))/9007199254740992 - (4872700232219253*sin(q1L))/9007199254740992))/36893488147419103232)))/36893488147419103232) - (7514214926474921*cos(q5L)*(((7514214926474921*cos(q4L))/36893488147419103232 + (4503599440548691*sin(q4L))/4503599627370496)*((9007199067919185*sin(q3L)*((56594998190739085871744456992395*cos(q1L))/81129638414606681695789005144064 - (43889380989894851923989405068805*sin(q1L))/81129638414606681695789005144064 + 63594381400292563045725890951477/664613997892457936451903530140172288))/9007199254740992 + cos(q3L)*((76229820211215127867025072518845*sin(q2L))/162259276829213363391578010288128 + cos(q2L)*((4872700232219253*cos(q1L))/9007199254740992 + (6283307137322267*sin(q1L))/9007199254740992) - (7514214926474921*sin(q2L)*((6283307137322267*cos(q1L))/9007199254740992 - (4872700232219253*sin(q1L))/9007199254740992))/36893488147419103232) + (7514214926474921*sin(q3L)*((7514214926474921*cos(q2L)*((6283307137322267*cos(q1L))/9007199254740992 - (4872700232219253*sin(q1L))/9007199254740992))/36893488147419103232 - (76229820211215127867025072518845*cos(q2L))/162259276829213363391578010288128 + sin(q2L)*((4872700232219253*cos(q1L))/9007199254740992 + (6283307137322267*sin(q1L))/9007199254740992)))/36893488147419103232) - ((9007199067919185*cos(q4L))/9007199254740992 - (234819211581865*sin(q4L))/1152921504606846976)*((425266980168672787164801917791314326747055225795*cos(q1L))/2993155353253689176481146537402947624255349848014848 + (686617165554103949950999710565799465200849541325*cos(q2L))/1461501637330902918203684832716283019655932542976 - (329794241748012540206902858004467560228111939405*sin(q1L))/2993155353253689176481146537402947624255349848014848 - (67682029681889335677290557259385*cos(q2L)*((6283307137322267*cos(q1L))/9007199254740992 - (4872700232219253*sin(q1L))/9007199254740992))/332306998946228968225951765070086144 - (9007199067919185*sin(q2L)*((4872700232219253*cos(q1L))/9007199254740992 + (6283307137322267*sin(q1L))/9007199254740992))/9007199254740992 + 477861849958017465213997854626476001002268408317/24519928653854221733733552434404946937899825954937634816) + (7514214926474921*sin(q4L)*((9007199067919185*cos(q3L)*((56594998190739085871744456992395*cos(q1L))/81129638414606681695789005144064 - (43889380989894851923989405068805*sin(q1L))/81129638414606681695789005144064 + 63594381400292563045725890951477/664613997892457936451903530140172288))/9007199254740992 + (7514214926474921*cos(q3L)*((7514214926474921*cos(q2L)*((6283307137322267*cos(q1L))/9007199254740992 - (4872700232219253*sin(q1L))/9007199254740992))/36893488147419103232 - (76229820211215127867025072518845*cos(q2L))/162259276829213363391578010288128 + sin(q2L)*((4872700232219253*cos(q1L))/9007199254740992 + (6283307137322267*sin(q1L))/9007199254740992)))/36893488147419103232 - sin(q3L)*((76229820211215127867025072518845*sin(q2L))/162259276829213363391578010288128 + cos(q2L)*((4872700232219253*cos(q1L))/9007199254740992 + (6283307137322267*sin(q1L))/9007199254740992) - (7514214926474921*sin(q2L)*((6283307137322267*cos(q1L))/9007199254740992 - (4872700232219253*sin(q1L))/9007199254740992))/36893488147419103232)))/36893488147419103232))/36893488147419103232))/36893488147419103232000 - (608651409044468601*cos(q4L)*((9007199067919185*cos(q3L)*((56594998190739085871744456992395*cos(q1L))/81129638414606681695789005144064 - (43889380989894851923989405068805*sin(q1L))/81129638414606681695789005144064 + 63594381400292563045725890951477/664613997892457936451903530140172288))/9007199254740992 + (7514214926474921*cos(q3L)*((7514214926474921*cos(q2L)*((6283307137322267*cos(q1L))/9007199254740992 - (4872700232219253*sin(q1L))/9007199254740992))/36893488147419103232 - (76229820211215127867025072518845*cos(q2L))/162259276829213363391578010288128 + sin(q2L)*((4872700232219253*cos(q1L))/9007199254740992 + (6283307137322267*sin(q1L))/9007199254740992)))/36893488147419103232 - sin(q3L)*((76229820211215127867025072518845*sin(q2L))/162259276829213363391578010288128 + cos(q2L)*((4872700232219253*cos(q1L))/9007199254740992 + (6283307137322267*sin(q1L))/9007199254740992) - (7514214926474921*sin(q2L)*((6283307137322267*cos(q1L))/9007199254740992 - (4872700232219253*sin(q1L))/9007199254740992))/36893488147419103232)))/73786976294838206464000 + (610321541873521657855151997354401418608858870661075444886782706002880706727*sin(q4L)*((9007199067919185*cos(q3L)*((56594998190739085871744456992395*cos(q1L))/81129638414606681695789005144064 - (43889380989894851923989405068805*sin(q1L))/81129638414606681695789005144064 + 63594381400292563045725890951477/664613997892457936451903530140172288))/9007199254740992 + (7514214926474921*cos(q3L)*((7514214926474921*cos(q2L)*((6283307137322267*cos(q1L))/9007199254740992 - (4872700232219253*sin(q1L))/9007199254740992))/36893488147419103232 - (76229820211215127867025072518845*cos(q2L))/162259276829213363391578010288128 + sin(q2L)*((4872700232219253*cos(q1L))/9007199254740992 + (6283307137322267*sin(q1L))/9007199254740992)))/36893488147419103232 - sin(q3L)*((76229820211215127867025072518845*sin(q2L))/162259276829213363391578010288128 + cos(q2L)*((4872700232219253*cos(q1L))/9007199254740992 + (6283307137322267*sin(q1L))/9007199254740992) - (7514214926474921*sin(q2L)*((6283307137322267*cos(q1L))/9007199254740992 - (4872700232219253*sin(q1L))/9007199254740992))/36893488147419103232)))/11307821214581659709333104004754678501295896940003961331978279688272766566400000 + (584133382113593486367040631332731*cos(q6L)*((9007199067919185*((7514214926474921*cos(q4L))/36893488147419103232 + (4503599440548691*sin(q4L))/4503599627370496)*((9007199067919185*sin(q3L)*((56594998190739085871744456992395*cos(q1L))/81129638414606681695789005144064 - (43889380989894851923989405068805*sin(q1L))/81129638414606681695789005144064 + 63594381400292563045725890951477/664613997892457936451903530140172288))/9007199254740992 + cos(q3L)*((76229820211215127867025072518845*sin(q2L))/162259276829213363391578010288128 + cos(q2L)*((4872700232219253*cos(q1L))/9007199254740992 + (6283307137322267*sin(q1L))/9007199254740992) - (7514214926474921*sin(q2L)*((6283307137322267*cos(q1L))/9007199254740992 - (4872700232219253*sin(q1L))/9007199254740992))/36893488147419103232) + (7514214926474921*sin(q3L)*((7514214926474921*cos(q2L)*((6283307137322267*cos(q1L))/9007199254740992 - (4872700232219253*sin(q1L))/9007199254740992))/36893488147419103232 - (76229820211215127867025072518845*cos(q2L))/162259276829213363391578010288128 + sin(q2L)*((4872700232219253*cos(q1L))/9007199254740992 + (6283307137322267*sin(q1L))/9007199254740992)))/36893488147419103232))/9007199254740992 - (9007199067919185*((9007199067919185*cos(q4L))/9007199254740992 - (234819211581865*sin(q4L))/1152921504606846976)*((425266980168672787164801917791314326747055225795*cos(q1L))/2993155353253689176481146537402947624255349848014848 + (686617165554103949950999710565799465200849541325*cos(q2L))/1461501637330902918203684832716283019655932542976 - (329794241748012540206902858004467560228111939405*sin(q1L))/2993155353253689176481146537402947624255349848014848 - (67682029681889335677290557259385*cos(q2L)*((6283307137322267*cos(q1L))/9007199254740992 - (4872700232219253*sin(q1L))/9007199254740992))/332306998946228968225951765070086144 - (9007199067919185*sin(q2L)*((4872700232219253*cos(q1L))/9007199254740992 + (6283307137322267*sin(q1L))/9007199254740992))/9007199254740992 + 477861849958017465213997854626476001002268408317/24519928653854221733733552434404946937899825954937634816))/9007199254740992 + (67682029681889335677290557259385*sin(q4L)*((9007199067919185*cos(q3L)*((56594998190739085871744456992395*cos(q1L))/81129638414606681695789005144064 - (43889380989894851923989405068805*sin(q1L))/81129638414606681695789005144064 + 63594381400292563045725890951477/664613997892457936451903530140172288))/9007199254740992 + (7514214926474921*cos(q3L)*((7514214926474921*cos(q2L)*((6283307137322267*cos(q1L))/9007199254740992 - (4872700232219253*sin(q1L))/9007199254740992))/36893488147419103232 - (76229820211215127867025072518845*cos(q2L))/162259276829213363391578010288128 + sin(q2L)*((4872700232219253*cos(q1L))/9007199254740992 + (6283307137322267*sin(q1L))/9007199254740992)))/36893488147419103232 - sin(q3L)*((76229820211215127867025072518845*sin(q2L))/162259276829213363391578010288128 + cos(q2L)*((4872700232219253*cos(q1L))/9007199254740992 + (6283307137322267*sin(q1L))/9007199254740992) - (7514214926474921*sin(q2L)*((6283307137322267*cos(q1L))/9007199254740992 - (4872700232219253*sin(q1L))/9007199254740992))/36893488147419103232)))/332306998946228968225951765070086144))/16225927682921336339157801028812800 + (48638874966763599*sin(q6L)*((9007199067919185*((7514214926474921*cos(q4L))/36893488147419103232 + (4503599440548691*sin(q4L))/4503599627370496)*((9007199067919185*sin(q3L)*((56594998190739085871744456992395*cos(q1L))/81129638414606681695789005144064 - (43889380989894851923989405068805*sin(q1L))/81129638414606681695789005144064 + 63594381400292563045725890951477/664613997892457936451903530140172288))/9007199254740992 + cos(q3L)*((76229820211215127867025072518845*sin(q2L))/162259276829213363391578010288128 + cos(q2L)*((4872700232219253*cos(q1L))/9007199254740992 + (6283307137322267*sin(q1L))/9007199254740992) - (7514214926474921*sin(q2L)*((6283307137322267*cos(q1L))/9007199254740992 - (4872700232219253*sin(q1L))/9007199254740992))/36893488147419103232) + (7514214926474921*sin(q3L)*((7514214926474921*cos(q2L)*((6283307137322267*cos(q1L))/9007199254740992 - (4872700232219253*sin(q1L))/9007199254740992))/36893488147419103232 - (76229820211215127867025072518845*cos(q2L))/162259276829213363391578010288128 + sin(q2L)*((4872700232219253*cos(q1L))/9007199254740992 + (6283307137322267*sin(q1L))/9007199254740992)))/36893488147419103232))/9007199254740992 - (9007199067919185*((9007199067919185*cos(q4L))/9007199254740992 - (234819211581865*sin(q4L))/1152921504606846976)*((425266980168672787164801917791314326747055225795*cos(q1L))/2993155353253689176481146537402947624255349848014848 + (686617165554103949950999710565799465200849541325*cos(q2L))/1461501637330902918203684832716283019655932542976 - (329794241748012540206902858004467560228111939405*sin(q1L))/2993155353253689176481146537402947624255349848014848 - (67682029681889335677290557259385*cos(q2L)*((6283307137322267*cos(q1L))/9007199254740992 - (4872700232219253*sin(q1L))/9007199254740992))/332306998946228968225951765070086144 - (9007199067919185*sin(q2L)*((4872700232219253*cos(q1L))/9007199254740992 + (6283307137322267*sin(q1L))/9007199254740992))/9007199254740992 + 477861849958017465213997854626476001002268408317/24519928653854221733733552434404946937899825954937634816))/9007199254740992 + (67682029681889335677290557259385*sin(q4L)*((9007199067919185*cos(q3L)*((56594998190739085871744456992395*cos(q1L))/81129638414606681695789005144064 - (43889380989894851923989405068805*sin(q1L))/81129638414606681695789005144064 + 63594381400292563045725890951477/664613997892457936451903530140172288))/9007199254740992 + (7514214926474921*cos(q3L)*((7514214926474921*cos(q2L)*((6283307137322267*cos(q1L))/9007199254740992 - (4872700232219253*sin(q1L))/9007199254740992))/36893488147419103232 - (76229820211215127867025072518845*cos(q2L))/162259276829213363391578010288128 + sin(q2L)*((4872700232219253*cos(q1L))/9007199254740992 + (6283307137322267*sin(q1L))/9007199254740992)))/36893488147419103232 - sin(q3L)*((76229820211215127867025072518845*sin(q2L))/162259276829213363391578010288128 + cos(q2L)*((4872700232219253*cos(q1L))/9007199254740992 + (6283307137322267*sin(q1L))/9007199254740992) - (7514214926474921*sin(q2L)*((6283307137322267*cos(q1L))/9007199254740992 - (4872700232219253*sin(q1L))/9007199254740992))/36893488147419103232)))/332306998946228968225951765070086144))/1801439850948198400, (48638874966763599*cos(q5L)*((666467732349846997487583938718911583194406904318712922873589125*cos(q1L))/113078212145816597093331040047546785012958969400039613319782796882727665664 + (1076049180065244948668759145796765391250102872519935285209856875*cos(q2L))/55213970774324510299478046898216203619608871777363092441300193790394368 - (516845254133432670685844229576986303733782399690601453662320875*sin(q1L))/113078212145816597093331040047546785012958969400039613319782796882727665664 - (81129635049124235038645691064225*cos(q3L)*((56594998190739085871744456992395*cos(q1L))/81129638414606681695789005144064 - (43889380989894851923989405068805*sin(q1L))/81129638414606681695789005144064 + 63594381400292563045725890951477/664613997892457936451903530140172288))/81129638414606681695789005144064 + (2115063383689692319117831580025*sin(q3L)*((56594998190739085871744456992395*cos(q1L))/81129638414606681695789005144064 - (43889380989894851923989405068805*sin(q1L))/81129638414606681695789005144064 + 63594381400292563045725890951477/664613997892457936451903530140172288))/10384593717069655257060992658440192 - (67682029681889335677290557259385*cos(q3L)*((7514214926474921*cos(q2L)*((6283307137322267*cos(q1L))/9007199254740992 - (4872700232219253*sin(q1L))/9007199254740992))/36893488147419103232 - (76229820211215127867025072518845*cos(q2L))/162259276829213363391578010288128 + sin(q2L)*((4872700232219253*cos(q1L))/9007199254740992 + (6283307137322267*sin(q1L))/9007199254740992)))/332306998946228968225951765070086144 + (234819211581865*cos(q3L)*((76229820211215127867025072518845*sin(q2L))/162259276829213363391578010288128 + cos(q2L)*((4872700232219253*cos(q1L))/9007199254740992 + (6283307137322267*sin(q1L))/9007199254740992) - (7514214926474921*sin(q2L)*((6283307137322267*cos(q1L))/9007199254740992 - (4872700232219253*sin(q1L))/9007199254740992))/36893488147419103232))/1152921504606846976 + (1764482024691522628700660907665*sin(q3L)*((7514214926474921*cos(q2L)*((6283307137322267*cos(q1L))/9007199254740992 - (4872700232219253*sin(q1L))/9007199254740992))/36893488147419103232 - (76229820211215127867025072518845*cos(q2L))/162259276829213363391578010288128 + sin(q2L)*((4872700232219253*cos(q1L))/9007199254740992 + (6283307137322267*sin(q1L))/9007199254740992)))/42535295865117307932921825928971026432 + (9007199067919185*sin(q3L)*((76229820211215127867025072518845*sin(q2L))/162259276829213363391578010288128 + cos(q2L)*((4872700232219253*cos(q1L))/9007199254740992 + (6283307137322267*sin(q1L))/9007199254740992) - (7514214926474921*sin(q2L)*((6283307137322267*cos(q1L))/9007199254740992 - (4872700232219253*sin(q1L))/9007199254740992))/36893488147419103232))/9007199254740992 - (106069577339469832923929692356850887620017617375*cos(q2L)*((6283307137322267*cos(q1L))/9007199254740992 - (4872700232219253*sin(q1L))/9007199254740992))/12554203470773361527671578846415332832204710888928069025792 - (14115856197532180673579726082375*sin(q2L)*((4872700232219253*cos(q1L))/9007199254740992 + (6283307137322267*sin(q1L))/9007199254740992))/340282366920938463463374607431768211456 + 748893091562634003789577347105888574211761174637088840996300475/926336713898529563388567880069503262826159877325124512315660672063305037119488))/1801439850948198400 + (170695144106365826517608855445768431563113584343*sin(q5L)*((666467732349846997487583938718911583194406904318712922873589125*cos(q1L))/113078212145816597093331040047546785012958969400039613319782796882727665664 + (1076049180065244948668759145796765391250102872519935285209856875*cos(q2L))/55213970774324510299478046898216203619608871777363092441300193790394368 - (516845254133432670685844229576986303733782399690601453662320875*sin(q1L))/113078212145816597093331040047546785012958969400039613319782796882727665664 - (81129635049124235038645691064225*cos(q3L)*((56594998190739085871744456992395*cos(q1L))/81129638414606681695789005144064 - (43889380989894851923989405068805*sin(q1L))/81129638414606681695789005144064 + 63594381400292563045725890951477/664613997892457936451903530140172288))/81129638414606681695789005144064 + (2115063383689692319117831580025*sin(q3L)*((56594998190739085871744456992395*cos(q1L))/81129638414606681695789005144064 - (43889380989894851923989405068805*sin(q1L))/81129638414606681695789005144064 + 63594381400292563045725890951477/664613997892457936451903530140172288))/10384593717069655257060992658440192 - (67682029681889335677290557259385*cos(q3L)*((7514214926474921*cos(q2L)*((6283307137322267*cos(q1L))/9007199254740992 - (4872700232219253*sin(q1L))/9007199254740992))/36893488147419103232 - (76229820211215127867025072518845*cos(q2L))/162259276829213363391578010288128 + sin(q2L)*((4872700232219253*cos(q1L))/9007199254740992 + (6283307137322267*sin(q1L))/9007199254740992)))/332306998946228968225951765070086144 + (234819211581865*cos(q3L)*((76229820211215127867025072518845*sin(q2L))/162259276829213363391578010288128 + cos(q2L)*((4872700232219253*cos(q1L))/9007199254740992 + (6283307137322267*sin(q1L))/9007199254740992) - (7514214926474921*sin(q2L)*((6283307137322267*cos(q1L))/9007199254740992 - (4872700232219253*sin(q1L))/9007199254740992))/36893488147419103232))/1152921504606846976 + (1764482024691522628700660907665*sin(q3L)*((7514214926474921*cos(q2L)*((6283307137322267*cos(q1L))/9007199254740992 - (4872700232219253*sin(q1L))/9007199254740992))/36893488147419103232 - (76229820211215127867025072518845*cos(q2L))/162259276829213363391578010288128 + sin(q2L)*((4872700232219253*cos(q1L))/9007199254740992 + (6283307137322267*sin(q1L))/9007199254740992)))/42535295865117307932921825928971026432 + (9007199067919185*sin(q3L)*((76229820211215127867025072518845*sin(q2L))/162259276829213363391578010288128 + cos(q2L)*((4872700232219253*cos(q1L))/9007199254740992 + (6283307137322267*sin(q1L))/9007199254740992) - (7514214926474921*sin(q2L)*((6283307137322267*cos(q1L))/9007199254740992 - (4872700232219253*sin(q1L))/9007199254740992))/36893488147419103232))/9007199254740992 - (106069577339469832923929692356850887620017617375*cos(q2L)*((6283307137322267*cos(q1L))/9007199254740992 - (4872700232219253*sin(q1L))/9007199254740992))/12554203470773361527671578846415332832204710888928069025792 - (14115856197532180673579726082375*sin(q2L)*((4872700232219253*cos(q1L))/9007199254740992 + (6283307137322267*sin(q1L))/9007199254740992))/340282366920938463463374607431768211456 + 748893091562634003789577347105888574211761174637088840996300475/926336713898529563388567880069503262826159877325124512315660672063305037119488))/119726214130147567059245861496117904970213993920593920 - (202883803014822867*cos(q5L)*(((4503599440548691*cos(q4L))/4503599627370496 - (7514214926474921*sin(q4L))/36893488147419103232)*((9007199067919185*sin(q3L)*((56594998190739085871744456992395*cos(q1L))/81129638414606681695789005144064 - (43889380989894851923989405068805*sin(q1L))/81129638414606681695789005144064 + 63594381400292563045725890951477/664613997892457936451903530140172288))/9007199254740992 + cos(q3L)*((76229820211215127867025072518845*sin(q2L))/162259276829213363391578010288128 + cos(q2L)*((4872700232219253*cos(q1L))/9007199254740992 + (6283307137322267*sin(q1L))/9007199254740992) - (7514214926474921*sin(q2L)*((6283307137322267*cos(q1L))/9007199254740992 - (4872700232219253*sin(q1L))/9007199254740992))/36893488147419103232) + (7514214926474921*sin(q3L)*((7514214926474921*cos(q2L)*((6283307137322267*cos(q1L))/9007199254740992 - (4872700232219253*sin(q1L))/9007199254740992))/36893488147419103232 - (76229820211215127867025072518845*cos(q2L))/162259276829213363391578010288128 + sin(q2L)*((4872700232219253*cos(q1L))/9007199254740992 + (6283307137322267*sin(q1L))/9007199254740992)))/36893488147419103232) + ((234819211581865*cos(q4L))/1152921504606846976 + (9007199067919185*sin(q4L))/9007199254740992)*((425266980168672787164801917791314326747055225795*cos(q1L))/2993155353253689176481146537402947624255349848014848 + (686617165554103949950999710565799465200849541325*cos(q2L))/1461501637330902918203684832716283019655932542976 - (329794241748012540206902858004467560228111939405*sin(q1L))/2993155353253689176481146537402947624255349848014848 - (67682029681889335677290557259385*cos(q2L)*((6283307137322267*cos(q1L))/9007199254740992 - (4872700232219253*sin(q1L))/9007199254740992))/332306998946228968225951765070086144 - (9007199067919185*sin(q2L)*((4872700232219253*cos(q1L))/9007199254740992 + (6283307137322267*sin(q1L))/9007199254740992))/9007199254740992 + 477861849958017465213997854626476001002268408317/24519928653854221733733552434404946937899825954937634816) + (7514214926474921*cos(q4L)*((9007199067919185*cos(q3L)*((56594998190739085871744456992395*cos(q1L))/81129638414606681695789005144064 - (43889380989894851923989405068805*sin(q1L))/81129638414606681695789005144064 + 63594381400292563045725890951477/664613997892457936451903530140172288))/9007199254740992 + (7514214926474921*cos(q3L)*((7514214926474921*cos(q2L)*((6283307137322267*cos(q1L))/9007199254740992 - (4872700232219253*sin(q1L))/9007199254740992))/36893488147419103232 - (76229820211215127867025072518845*cos(q2L))/162259276829213363391578010288128 + sin(q2L)*((4872700232219253*cos(q1L))/9007199254740992 + (6283307137322267*sin(q1L))/9007199254740992)))/36893488147419103232 - sin(q3L)*((76229820211215127867025072518845*sin(q2L))/162259276829213363391578010288128 + cos(q2L)*((4872700232219253*cos(q1L))/9007199254740992 + (6283307137322267*sin(q1L))/9007199254740992) - (7514214926474921*sin(q2L)*((6283307137322267*cos(q1L))/9007199254740992 - (4872700232219253*sin(q1L))/9007199254740992))/36893488147419103232)))/36893488147419103232))/36893488147419103232000 - (712008244765680093343103025701132101054572137019*sin(q5L)*(((4503599440548691*cos(q4L))/4503599627370496 - (7514214926474921*sin(q4L))/36893488147419103232)*((9007199067919185*sin(q3L)*((56594998190739085871744456992395*cos(q1L))/81129638414606681695789005144064 - (43889380989894851923989405068805*sin(q1L))/81129638414606681695789005144064 + 63594381400292563045725890951477/664613997892457936451903530140172288))/9007199254740992 + cos(q3L)*((76229820211215127867025072518845*sin(q2L))/162259276829213363391578010288128 + cos(q2L)*((4872700232219253*cos(q1L))/9007199254740992 + (6283307137322267*sin(q1L))/9007199254740992) - (7514214926474921*sin(q2L)*((6283307137322267*cos(q1L))/9007199254740992 - (4872700232219253*sin(q1L))/9007199254740992))/36893488147419103232) + (7514214926474921*sin(q3L)*((7514214926474921*cos(q2L)*((6283307137322267*cos(q1L))/9007199254740992 - (4872700232219253*sin(q1L))/9007199254740992))/36893488147419103232 - (76229820211215127867025072518845*cos(q2L))/162259276829213363391578010288128 + sin(q2L)*((4872700232219253*cos(q1L))/9007199254740992 + (6283307137322267*sin(q1L))/9007199254740992)))/36893488147419103232) + ((234819211581865*cos(q4L))/1152921504606846976 + (9007199067919185*sin(q4L))/9007199254740992)*((425266980168672787164801917791314326747055225795*cos(q1L))/2993155353253689176481146537402947624255349848014848 + (686617165554103949950999710565799465200849541325*cos(q2L))/1461501637330902918203684832716283019655932542976 - (329794241748012540206902858004467560228111939405*sin(q1L))/2993155353253689176481146537402947624255349848014848 - (67682029681889335677290557259385*cos(q2L)*((6283307137322267*cos(q1L))/9007199254740992 - (4872700232219253*sin(q1L))/9007199254740992))/332306998946228968225951765070086144 - (9007199067919185*sin(q2L)*((4872700232219253*cos(q1L))/9007199254740992 + (6283307137322267*sin(q1L))/9007199254740992))/9007199254740992 + 477861849958017465213997854626476001002268408317/24519928653854221733733552434404946937899825954937634816) + (7514214926474921*cos(q4L)*((9007199067919185*cos(q3L)*((56594998190739085871744456992395*cos(q1L))/81129638414606681695789005144064 - (43889380989894851923989405068805*sin(q1L))/81129638414606681695789005144064 + 63594381400292563045725890951477/664613997892457936451903530140172288))/9007199254740992 + (7514214926474921*cos(q3L)*((7514214926474921*cos(q2L)*((6283307137322267*cos(q1L))/9007199254740992 - (4872700232219253*sin(q1L))/9007199254740992))/36893488147419103232 - (76229820211215127867025072518845*cos(q2L))/162259276829213363391578010288128 + sin(q2L)*((4872700232219253*cos(q1L))/9007199254740992 + (6283307137322267*sin(q1L))/9007199254740992)))/36893488147419103232 - sin(q3L)*((76229820211215127867025072518845*sin(q2L))/162259276829213363391578010288128 + cos(q2L)*((4872700232219253*cos(q1L))/9007199254740992 + (6283307137322267*sin(q1L))/9007199254740992) - (7514214926474921*sin(q2L)*((6283307137322267*cos(q1L))/9007199254740992 - (4872700232219253*sin(q1L))/9007199254740992))/36893488147419103232)))/36893488147419103232))/2451992865385422173373355243440494693789982595493763481600 + (94754841554645069948206780163139*cos(q5L)*(((7514214926474921*cos(q4L))/36893488147419103232 + (4503599440548691*sin(q4L))/4503599627370496)*((9007199067919185*sin(q3L)*((56594998190739085871744456992395*cos(q1L))/81129638414606681695789005144064 - (43889380989894851923989405068805*sin(q1L))/81129638414606681695789005144064 + 63594381400292563045725890951477/664613997892457936451903530140172288))/9007199254740992 + cos(q3L)*((76229820211215127867025072518845*sin(q2L))/162259276829213363391578010288128 + cos(q2L)*((4872700232219253*cos(q1L))/9007199254740992 + (6283307137322267*sin(q1L))/9007199254740992) - (7514214926474921*sin(q2L)*((6283307137322267*cos(q1L))/9007199254740992 - (4872700232219253*sin(q1L))/9007199254740992))/36893488147419103232) + (7514214926474921*sin(q3L)*((7514214926474921*cos(q2L)*((6283307137322267*cos(q1L))/9007199254740992 - (4872700232219253*sin(q1L))/9007199254740992))/36893488147419103232 - (76229820211215127867025072518845*cos(q2L))/162259276829213363391578010288128 + sin(q2L)*((4872700232219253*cos(q1L))/9007199254740992 + (6283307137322267*sin(q1L))/9007199254740992)))/36893488147419103232) - ((9007199067919185*cos(q4L))/9007199254740992 - (234819211581865*sin(q4L))/1152921504606846976)*((425266980168672787164801917791314326747055225795*cos(q1L))/2993155353253689176481146537402947624255349848014848 + (686617165554103949950999710565799465200849541325*cos(q2L))/1461501637330902918203684832716283019655932542976 - (329794241748012540206902858004467560228111939405*sin(q1L))/2993155353253689176481146537402947624255349848014848 - (67682029681889335677290557259385*cos(q2L)*((6283307137322267*cos(q1L))/9007199254740992 - (4872700232219253*sin(q1L))/9007199254740992))/332306998946228968225951765070086144 - (9007199067919185*sin(q2L)*((4872700232219253*cos(q1L))/9007199254740992 + (6283307137322267*sin(q1L))/9007199254740992))/9007199254740992 + 477861849958017465213997854626476001002268408317/24519928653854221733733552434404946937899825954937634816) + (7514214926474921*sin(q4L)*((9007199067919185*cos(q3L)*((56594998190739085871744456992395*cos(q1L))/81129638414606681695789005144064 - (43889380989894851923989405068805*sin(q1L))/81129638414606681695789005144064 + 63594381400292563045725890951477/664613997892457936451903530140172288))/9007199254740992 + (7514214926474921*cos(q3L)*((7514214926474921*cos(q2L)*((6283307137322267*cos(q1L))/9007199254740992 - (4872700232219253*sin(q1L))/9007199254740992))/36893488147419103232 - (76229820211215127867025072518845*cos(q2L))/162259276829213363391578010288128 + sin(q2L)*((4872700232219253*cos(q1L))/9007199254740992 + (6283307137322267*sin(q1L))/9007199254740992)))/36893488147419103232 - sin(q3L)*((76229820211215127867025072518845*sin(q2L))/162259276829213363391578010288128 + cos(q2L)*((4872700232219253*cos(q1L))/9007199254740992 + (6283307137322267*sin(q1L))/9007199254740992) - (7514214926474921*sin(q2L)*((6283307137322267*cos(q1L))/9007199254740992 - (4872700232219253*sin(q1L))/9007199254740992))/36893488147419103232)))/36893488147419103232))/66461399789245793645190353014017228800 - (27*sin(q5L)*(((7514214926474921*cos(q4L))/36893488147419103232 + (4503599440548691*sin(q4L))/4503599627370496)*((9007199067919185*sin(q3L)*((56594998190739085871744456992395*cos(q1L))/81129638414606681695789005144064 - (43889380989894851923989405068805*sin(q1L))/81129638414606681695789005144064 + 63594381400292563045725890951477/664613997892457936451903530140172288))/9007199254740992 + cos(q3L)*((76229820211215127867025072518845*sin(q2L))/162259276829213363391578010288128 + cos(q2L)*((4872700232219253*cos(q1L))/9007199254740992 + (6283307137322267*sin(q1L))/9007199254740992) - (7514214926474921*sin(q2L)*((6283307137322267*cos(q1L))/9007199254740992 - (4872700232219253*sin(q1L))/9007199254740992))/36893488147419103232) + (7514214926474921*sin(q3L)*((7514214926474921*cos(q2L)*((6283307137322267*cos(q1L))/9007199254740992 - (4872700232219253*sin(q1L))/9007199254740992))/36893488147419103232 - (76229820211215127867025072518845*cos(q2L))/162259276829213363391578010288128 + sin(q2L)*((4872700232219253*cos(q1L))/9007199254740992 + (6283307137322267*sin(q1L))/9007199254740992)))/36893488147419103232) - ((9007199067919185*cos(q4L))/9007199254740992 - (234819211581865*sin(q4L))/1152921504606846976)*((425266980168672787164801917791314326747055225795*cos(q1L))/2993155353253689176481146537402947624255349848014848 + (686617165554103949950999710565799465200849541325*cos(q2L))/1461501637330902918203684832716283019655932542976 - (329794241748012540206902858004467560228111939405*sin(q1L))/2993155353253689176481146537402947624255349848014848 - (67682029681889335677290557259385*cos(q2L)*((6283307137322267*cos(q1L))/9007199254740992 - (4872700232219253*sin(q1L))/9007199254740992))/332306998946228968225951765070086144 - (9007199067919185*sin(q2L)*((4872700232219253*cos(q1L))/9007199254740992 + (6283307137322267*sin(q1L))/9007199254740992))/9007199254740992 + 477861849958017465213997854626476001002268408317/24519928653854221733733552434404946937899825954937634816) + (7514214926474921*sin(q4L)*((9007199067919185*cos(q3L)*((56594998190739085871744456992395*cos(q1L))/81129638414606681695789005144064 - (43889380989894851923989405068805*sin(q1L))/81129638414606681695789005144064 + 63594381400292563045725890951477/664613997892457936451903530140172288))/9007199254740992 + (7514214926474921*cos(q3L)*((7514214926474921*cos(q2L)*((6283307137322267*cos(q1L))/9007199254740992 - (4872700232219253*sin(q1L))/9007199254740992))/36893488147419103232 - (76229820211215127867025072518845*cos(q2L))/162259276829213363391578010288128 + sin(q2L)*((4872700232219253*cos(q1L))/9007199254740992 + (6283307137322267*sin(q1L))/9007199254740992)))/36893488147419103232 - sin(q3L)*((76229820211215127867025072518845*sin(q2L))/162259276829213363391578010288128 + cos(q2L)*((4872700232219253*cos(q1L))/9007199254740992 + (6283307137322267*sin(q1L))/9007199254740992) - (7514214926474921*sin(q2L)*((6283307137322267*cos(q1L))/9007199254740992 - (4872700232219253*sin(q1L))/9007199254740992))/36893488147419103232)))/36893488147419103232))/1000 + (27*cos(q6L)*((7514214926474921*cos(q5L)*(((4503599440548691*cos(q4L))/4503599627370496 - (7514214926474921*sin(q4L))/36893488147419103232)*((9007199067919185*sin(q3L)*((56594998190739085871744456992395*cos(q1L))/81129638414606681695789005144064 - (43889380989894851923989405068805*sin(q1L))/81129638414606681695789005144064 + 63594381400292563045725890951477/664613997892457936451903530140172288))/9007199254740992 + cos(q3L)*((76229820211215127867025072518845*sin(q2L))/162259276829213363391578010288128 + cos(q2L)*((4872700232219253*cos(q1L))/9007199254740992 + (6283307137322267*sin(q1L))/9007199254740992) - (7514214926474921*sin(q2L)*((6283307137322267*cos(q1L))/9007199254740992 - (4872700232219253*sin(q1L))/9007199254740992))/36893488147419103232) + (7514214926474921*sin(q3L)*((7514214926474921*cos(q2L)*((6283307137322267*cos(q1L))/9007199254740992 - (4872700232219253*sin(q1L))/9007199254740992))/36893488147419103232 - (76229820211215127867025072518845*cos(q2L))/162259276829213363391578010288128 + sin(q2L)*((4872700232219253*cos(q1L))/9007199254740992 + (6283307137322267*sin(q1L))/9007199254740992)))/36893488147419103232) + ((234819211581865*cos(q4L))/1152921504606846976 + (9007199067919185*sin(q4L))/9007199254740992)*((425266980168672787164801917791314326747055225795*cos(q1L))/2993155353253689176481146537402947624255349848014848 + (686617165554103949950999710565799465200849541325*cos(q2L))/1461501637330902918203684832716283019655932542976 - (329794241748012540206902858004467560228111939405*sin(q1L))/2993155353253689176481146537402947624255349848014848 - (67682029681889335677290557259385*cos(q2L)*((6283307137322267*cos(q1L))/9007199254740992 - (4872700232219253*sin(q1L))/9007199254740992))/332306998946228968225951765070086144 - (9007199067919185*sin(q2L)*((4872700232219253*cos(q1L))/9007199254740992 + (6283307137322267*sin(q1L))/9007199254740992))/9007199254740992 + 477861849958017465213997854626476001002268408317/24519928653854221733733552434404946937899825954937634816) + (7514214926474921*cos(q4L)*((9007199067919185*cos(q3L)*((56594998190739085871744456992395*cos(q1L))/81129638414606681695789005144064 - (43889380989894851923989405068805*sin(q1L))/81129638414606681695789005144064 + 63594381400292563045725890951477/664613997892457936451903530140172288))/9007199254740992 + (7514214926474921*cos(q3L)*((7514214926474921*cos(q2L)*((6283307137322267*cos(q1L))/9007199254740992 - (4872700232219253*sin(q1L))/9007199254740992))/36893488147419103232 - (76229820211215127867025072518845*cos(q2L))/162259276829213363391578010288128 + sin(q2L)*((4872700232219253*cos(q1L))/9007199254740992 + (6283307137322267*sin(q1L))/9007199254740992)))/36893488147419103232 - sin(q3L)*((76229820211215127867025072518845*sin(q2L))/162259276829213363391578010288128 + cos(q2L)*((4872700232219253*cos(q1L))/9007199254740992 + (6283307137322267*sin(q1L))/9007199254740992) - (7514214926474921*sin(q2L)*((6283307137322267*cos(q1L))/9007199254740992 - (4872700232219253*sin(q1L))/9007199254740992))/36893488147419103232)))/36893488147419103232))/36893488147419103232 - (9007199067919185*cos(q5L)*((666467732349846997487583938718911583194406904318712922873589125*cos(q1L))/113078212145816597093331040047546785012958969400039613319782796882727665664 + (1076049180065244948668759145796765391250102872519935285209856875*cos(q2L))/55213970774324510299478046898216203619608871777363092441300193790394368 - (516845254133432670685844229576986303733782399690601453662320875*sin(q1L))/113078212145816597093331040047546785012958969400039613319782796882727665664 - (81129635049124235038645691064225*cos(q3L)*((56594998190739085871744456992395*cos(q1L))/81129638414606681695789005144064 - (43889380989894851923989405068805*sin(q1L))/81129638414606681695789005144064 + 63594381400292563045725890951477/664613997892457936451903530140172288))/81129638414606681695789005144064 + (2115063383689692319117831580025*sin(q3L)*((56594998190739085871744456992395*cos(q1L))/81129638414606681695789005144064 - (43889380989894851923989405068805*sin(q1L))/81129638414606681695789005144064 + 63594381400292563045725890951477/664613997892457936451903530140172288))/10384593717069655257060992658440192 - (67682029681889335677290557259385*cos(q3L)*((7514214926474921*cos(q2L)*((6283307137322267*cos(q1L))/9007199254740992 - (4872700232219253*sin(q1L))/9007199254740992))/36893488147419103232 - (76229820211215127867025072518845*cos(q2L))/162259276829213363391578010288128 + sin(q2L)*((4872700232219253*cos(q1L))/9007199254740992 + (6283307137322267*sin(q1L))/9007199254740992)))/332306998946228968225951765070086144 + (234819211581865*cos(q3L)*((76229820211215127867025072518845*sin(q2L))/162259276829213363391578010288128 + cos(q2L)*((4872700232219253*cos(q1L))/9007199254740992 + (6283307137322267*sin(q1L))/9007199254740992) - (7514214926474921*sin(q2L)*((6283307137322267*cos(q1L))/9007199254740992 - (4872700232219253*sin(q1L))/9007199254740992))/36893488147419103232))/1152921504606846976 + (1764482024691522628700660907665*sin(q3L)*((7514214926474921*cos(q2L)*((6283307137322267*cos(q1L))/9007199254740992 - (4872700232219253*sin(q1L))/9007199254740992))/36893488147419103232 - (76229820211215127867025072518845*cos(q2L))/162259276829213363391578010288128 + sin(q2L)*((4872700232219253*cos(q1L))/9007199254740992 + (6283307137322267*sin(q1L))/9007199254740992)))/42535295865117307932921825928971026432 + (9007199067919185*sin(q3L)*((76229820211215127867025072518845*sin(q2L))/162259276829213363391578010288128 + cos(q2L)*((4872700232219253*cos(q1L))/9007199254740992 + (6283307137322267*sin(q1L))/9007199254740992) - (7514214926474921*sin(q2L)*((6283307137322267*cos(q1L))/9007199254740992 - (4872700232219253*sin(q1L))/9007199254740992))/36893488147419103232))/9007199254740992 - (106069577339469832923929692356850887620017617375*cos(q2L)*((6283307137322267*cos(q1L))/9007199254740992 - (4872700232219253*sin(q1L))/9007199254740992))/12554203470773361527671578846415332832204710888928069025792 - (14115856197532180673579726082375*sin(q2L)*((4872700232219253*cos(q1L))/9007199254740992 + (6283307137322267*sin(q1L))/9007199254740992))/340282366920938463463374607431768211456 + 748893091562634003789577347105888574211761174637088840996300475/926336713898529563388567880069503262826159877325124512315660672063305037119488))/9007199254740992 + sin(q5L)*(((7514214926474921*cos(q4L))/36893488147419103232 + (4503599440548691*sin(q4L))/4503599627370496)*((9007199067919185*sin(q3L)*((56594998190739085871744456992395*cos(q1L))/81129638414606681695789005144064 - (43889380989894851923989405068805*sin(q1L))/81129638414606681695789005144064 + 63594381400292563045725890951477/664613997892457936451903530140172288))/9007199254740992 + cos(q3L)*((76229820211215127867025072518845*sin(q2L))/162259276829213363391578010288128 + cos(q2L)*((4872700232219253*cos(q1L))/9007199254740992 + (6283307137322267*sin(q1L))/9007199254740992) - (7514214926474921*sin(q2L)*((6283307137322267*cos(q1L))/9007199254740992 - (4872700232219253*sin(q1L))/9007199254740992))/36893488147419103232) + (7514214926474921*sin(q3L)*((7514214926474921*cos(q2L)*((6283307137322267*cos(q1L))/9007199254740992 - (4872700232219253*sin(q1L))/9007199254740992))/36893488147419103232 - (76229820211215127867025072518845*cos(q2L))/162259276829213363391578010288128 + sin(q2L)*((4872700232219253*cos(q1L))/9007199254740992 + (6283307137322267*sin(q1L))/9007199254740992)))/36893488147419103232) - ((9007199067919185*cos(q4L))/9007199254740992 - (234819211581865*sin(q4L))/1152921504606846976)*((425266980168672787164801917791314326747055225795*cos(q1L))/2993155353253689176481146537402947624255349848014848 + (686617165554103949950999710565799465200849541325*cos(q2L))/1461501637330902918203684832716283019655932542976 - (329794241748012540206902858004467560228111939405*sin(q1L))/2993155353253689176481146537402947624255349848014848 - (67682029681889335677290557259385*cos(q2L)*((6283307137322267*cos(q1L))/9007199254740992 - (4872700232219253*sin(q1L))/9007199254740992))/332306998946228968225951765070086144 - (9007199067919185*sin(q2L)*((4872700232219253*cos(q1L))/9007199254740992 + (6283307137322267*sin(q1L))/9007199254740992))/9007199254740992 + 477861849958017465213997854626476001002268408317/24519928653854221733733552434404946937899825954937634816) + (7514214926474921*sin(q4L)*((9007199067919185*cos(q3L)*((56594998190739085871744456992395*cos(q1L))/81129638414606681695789005144064 - (43889380989894851923989405068805*sin(q1L))/81129638414606681695789005144064 + 63594381400292563045725890951477/664613997892457936451903530140172288))/9007199254740992 + (7514214926474921*cos(q3L)*((7514214926474921*cos(q2L)*((6283307137322267*cos(q1L))/9007199254740992 - (4872700232219253*sin(q1L))/9007199254740992))/36893488147419103232 - (76229820211215127867025072518845*cos(q2L))/162259276829213363391578010288128 + sin(q2L)*((4872700232219253*cos(q1L))/9007199254740992 + (6283307137322267*sin(q1L))/9007199254740992)))/36893488147419103232 - sin(q3L)*((76229820211215127867025072518845*sin(q2L))/162259276829213363391578010288128 + cos(q2L)*((4872700232219253*cos(q1L))/9007199254740992 + (6283307137322267*sin(q1L))/9007199254740992) - (7514214926474921*sin(q2L)*((6283307137322267*cos(q1L))/9007199254740992 - (4872700232219253*sin(q1L))/9007199254740992))/36893488147419103232)))/36893488147419103232)))/1000 - (2436553109258773196144549622003023*cos(q6L)*((9007199067919185*sin(q5L)*((666467732349846997487583938718911583194406904318712922873589125*cos(q1L))/113078212145816597093331040047546785012958969400039613319782796882727665664 + (1076049180065244948668759145796765391250102872519935285209856875*cos(q2L))/55213970774324510299478046898216203619608871777363092441300193790394368 - (516845254133432670685844229576986303733782399690601453662320875*sin(q1L))/113078212145816597093331040047546785012958969400039613319782796882727665664 - (81129635049124235038645691064225*cos(q3L)*((56594998190739085871744456992395*cos(q1L))/81129638414606681695789005144064 - (43889380989894851923989405068805*sin(q1L))/81129638414606681695789005144064 + 63594381400292563045725890951477/664613997892457936451903530140172288))/81129638414606681695789005144064 + (2115063383689692319117831580025*sin(q3L)*((56594998190739085871744456992395*cos(q1L))/81129638414606681695789005144064 - (43889380989894851923989405068805*sin(q1L))/81129638414606681695789005144064 + 63594381400292563045725890951477/664613997892457936451903530140172288))/10384593717069655257060992658440192 - (67682029681889335677290557259385*cos(q3L)*((7514214926474921*cos(q2L)*((6283307137322267*cos(q1L))/9007199254740992 - (4872700232219253*sin(q1L))/9007199254740992))/36893488147419103232 - (76229820211215127867025072518845*cos(q2L))/162259276829213363391578010288128 + sin(q2L)*((4872700232219253*cos(q1L))/9007199254740992 + (6283307137322267*sin(q1L))/9007199254740992)))/332306998946228968225951765070086144 + (234819211581865*cos(q3L)*((76229820211215127867025072518845*sin(q2L))/162259276829213363391578010288128 + cos(q2L)*((4872700232219253*cos(q1L))/9007199254740992 + (6283307137322267*sin(q1L))/9007199254740992) - (7514214926474921*sin(q2L)*((6283307137322267*cos(q1L))/9007199254740992 - (4872700232219253*sin(q1L))/9007199254740992))/36893488147419103232))/1152921504606846976 + (1764482024691522628700660907665*sin(q3L)*((7514214926474921*cos(q2L)*((6283307137322267*cos(q1L))/9007199254740992 - (4872700232219253*sin(q1L))/9007199254740992))/36893488147419103232 - (76229820211215127867025072518845*cos(q2L))/162259276829213363391578010288128 + sin(q2L)*((4872700232219253*cos(q1L))/9007199254740992 + (6283307137322267*sin(q1L))/9007199254740992)))/42535295865117307932921825928971026432 + (9007199067919185*sin(q3L)*((76229820211215127867025072518845*sin(q2L))/162259276829213363391578010288128 + cos(q2L)*((4872700232219253*cos(q1L))/9007199254740992 + (6283307137322267*sin(q1L))/9007199254740992) - (7514214926474921*sin(q2L)*((6283307137322267*cos(q1L))/9007199254740992 - (4872700232219253*sin(q1L))/9007199254740992))/36893488147419103232))/9007199254740992 - (106069577339469832923929692356850887620017617375*cos(q2L)*((6283307137322267*cos(q1L))/9007199254740992 - (4872700232219253*sin(q1L))/9007199254740992))/12554203470773361527671578846415332832204710888928069025792 - (14115856197532180673579726082375*sin(q2L)*((4872700232219253*cos(q1L))/9007199254740992 + (6283307137322267*sin(q1L))/9007199254740992))/340282366920938463463374607431768211456 + 748893091562634003789577347105888574211761174637088840996300475/926336713898529563388567880069503262826159877325124512315660672063305037119488))/9007199254740992 - (7514214926474921*sin(q5L)*(((4503599440548691*cos(q4L))/4503599627370496 - (7514214926474921*sin(q4L))/36893488147419103232)*((9007199067919185*sin(q3L)*((56594998190739085871744456992395*cos(q1L))/81129638414606681695789005144064 - (43889380989894851923989405068805*sin(q1L))/81129638414606681695789005144064 + 63594381400292563045725890951477/664613997892457936451903530140172288))/9007199254740992 + cos(q3L)*((76229820211215127867025072518845*sin(q2L))/162259276829213363391578010288128 + cos(q2L)*((4872700232219253*cos(q1L))/9007199254740992 + (6283307137322267*sin(q1L))/9007199254740992) - (7514214926474921*sin(q2L)*((6283307137322267*cos(q1L))/9007199254740992 - (4872700232219253*sin(q1L))/9007199254740992))/36893488147419103232) + (7514214926474921*sin(q3L)*((7514214926474921*cos(q2L)*((6283307137322267*cos(q1L))/9007199254740992 - (4872700232219253*sin(q1L))/9007199254740992))/36893488147419103232 - (76229820211215127867025072518845*cos(q2L))/162259276829213363391578010288128 + sin(q2L)*((4872700232219253*cos(q1L))/9007199254740992 + (6283307137322267*sin(q1L))/9007199254740992)))/36893488147419103232) + ((234819211581865*cos(q4L))/1152921504606846976 + (9007199067919185*sin(q4L))/9007199254740992)*((425266980168672787164801917791314326747055225795*cos(q1L))/2993155353253689176481146537402947624255349848014848 + (686617165554103949950999710565799465200849541325*cos(q2L))/1461501637330902918203684832716283019655932542976 - (329794241748012540206902858004467560228111939405*sin(q1L))/2993155353253689176481146537402947624255349848014848 - (67682029681889335677290557259385*cos(q2L)*((6283307137322267*cos(q1L))/9007199254740992 - (4872700232219253*sin(q1L))/9007199254740992))/332306998946228968225951765070086144 - (9007199067919185*sin(q2L)*((4872700232219253*cos(q1L))/9007199254740992 + (6283307137322267*sin(q1L))/9007199254740992))/9007199254740992 + 477861849958017465213997854626476001002268408317/24519928653854221733733552434404946937899825954937634816) + (7514214926474921*cos(q4L)*((9007199067919185*cos(q3L)*((56594998190739085871744456992395*cos(q1L))/81129638414606681695789005144064 - (43889380989894851923989405068805*sin(q1L))/81129638414606681695789005144064 + 63594381400292563045725890951477/664613997892457936451903530140172288))/9007199254740992 + (7514214926474921*cos(q3L)*((7514214926474921*cos(q2L)*((6283307137322267*cos(q1L))/9007199254740992 - (4872700232219253*sin(q1L))/9007199254740992))/36893488147419103232 - (76229820211215127867025072518845*cos(q2L))/162259276829213363391578010288128 + sin(q2L)*((4872700232219253*cos(q1L))/9007199254740992 + (6283307137322267*sin(q1L))/9007199254740992)))/36893488147419103232 - sin(q3L)*((76229820211215127867025072518845*sin(q2L))/162259276829213363391578010288128 + cos(q2L)*((4872700232219253*cos(q1L))/9007199254740992 + (6283307137322267*sin(q1L))/9007199254740992) - (7514214926474921*sin(q2L)*((6283307137322267*cos(q1L))/9007199254740992 - (4872700232219253*sin(q1L))/9007199254740992))/36893488147419103232)))/36893488147419103232))/36893488147419103232 + cos(q5L)*(((7514214926474921*cos(q4L))/36893488147419103232 + (4503599440548691*sin(q4L))/4503599627370496)*((9007199067919185*sin(q3L)*((56594998190739085871744456992395*cos(q1L))/81129638414606681695789005144064 - (43889380989894851923989405068805*sin(q1L))/81129638414606681695789005144064 + 63594381400292563045725890951477/664613997892457936451903530140172288))/9007199254740992 + cos(q3L)*((76229820211215127867025072518845*sin(q2L))/162259276829213363391578010288128 + cos(q2L)*((4872700232219253*cos(q1L))/9007199254740992 + (6283307137322267*sin(q1L))/9007199254740992) - (7514214926474921*sin(q2L)*((6283307137322267*cos(q1L))/9007199254740992 - (4872700232219253*sin(q1L))/9007199254740992))/36893488147419103232) + (7514214926474921*sin(q3L)*((7514214926474921*cos(q2L)*((6283307137322267*cos(q1L))/9007199254740992 - (4872700232219253*sin(q1L))/9007199254740992))/36893488147419103232 - (76229820211215127867025072518845*cos(q2L))/162259276829213363391578010288128 + sin(q2L)*((4872700232219253*cos(q1L))/9007199254740992 + (6283307137322267*sin(q1L))/9007199254740992)))/36893488147419103232) - ((9007199067919185*cos(q4L))/9007199254740992 - (234819211581865*sin(q4L))/1152921504606846976)*((425266980168672787164801917791314326747055225795*cos(q1L))/2993155353253689176481146537402947624255349848014848 + (686617165554103949950999710565799465200849541325*cos(q2L))/1461501637330902918203684832716283019655932542976 - (329794241748012540206902858004467560228111939405*sin(q1L))/2993155353253689176481146537402947624255349848014848 - (67682029681889335677290557259385*cos(q2L)*((6283307137322267*cos(q1L))/9007199254740992 - (4872700232219253*sin(q1L))/9007199254740992))/332306998946228968225951765070086144 - (9007199067919185*sin(q2L)*((4872700232219253*cos(q1L))/9007199254740992 + (6283307137322267*sin(q1L))/9007199254740992))/9007199254740992 + 477861849958017465213997854626476001002268408317/24519928653854221733733552434404946937899825954937634816) + (7514214926474921*sin(q4L)*((9007199067919185*cos(q3L)*((56594998190739085871744456992395*cos(q1L))/81129638414606681695789005144064 - (43889380989894851923989405068805*sin(q1L))/81129638414606681695789005144064 + 63594381400292563045725890951477/664613997892457936451903530140172288))/9007199254740992 + (7514214926474921*cos(q3L)*((7514214926474921*cos(q2L)*((6283307137322267*cos(q1L))/9007199254740992 - (4872700232219253*sin(q1L))/9007199254740992))/36893488147419103232 - (76229820211215127867025072518845*cos(q2L))/162259276829213363391578010288128 + sin(q2L)*((4872700232219253*cos(q1L))/9007199254740992 + (6283307137322267*sin(q1L))/9007199254740992)))/36893488147419103232 - sin(q3L)*((76229820211215127867025072518845*sin(q2L))/162259276829213363391578010288128 + cos(q2L)*((4872700232219253*cos(q1L))/9007199254740992 + (6283307137322267*sin(q1L))/9007199254740992) - (7514214926474921*sin(q2L)*((6283307137322267*cos(q1L))/9007199254740992 - (4872700232219253*sin(q1L))/9007199254740992))/36893488147419103232)))/36893488147419103232)))/332306998946228968225951765070086144000 - (324259171862923063*sin(q6L)*((7514214926474921*cos(q5L)*(((4503599440548691*cos(q4L))/4503599627370496 - (7514214926474921*sin(q4L))/36893488147419103232)*((9007199067919185*sin(q3L)*((56594998190739085871744456992395*cos(q1L))/81129638414606681695789005144064 - (43889380989894851923989405068805*sin(q1L))/81129638414606681695789005144064 + 63594381400292563045725890951477/664613997892457936451903530140172288))/9007199254740992 + cos(q3L)*((76229820211215127867025072518845*sin(q2L))/162259276829213363391578010288128 + cos(q2L)*((4872700232219253*cos(q1L))/9007199254740992 + (6283307137322267*sin(q1L))/9007199254740992) - (7514214926474921*sin(q2L)*((6283307137322267*cos(q1L))/9007199254740992 - (4872700232219253*sin(q1L))/9007199254740992))/36893488147419103232) + (7514214926474921*sin(q3L)*((7514214926474921*cos(q2L)*((6283307137322267*cos(q1L))/9007199254740992 - (4872700232219253*sin(q1L))/9007199254740992))/36893488147419103232 - (76229820211215127867025072518845*cos(q2L))/162259276829213363391578010288128 + sin(q2L)*((4872700232219253*cos(q1L))/9007199254740992 + (6283307137322267*sin(q1L))/9007199254740992)))/36893488147419103232) + ((234819211581865*cos(q4L))/1152921504606846976 + (9007199067919185*sin(q4L))/9007199254740992)*((425266980168672787164801917791314326747055225795*cos(q1L))/2993155353253689176481146537402947624255349848014848 + (686617165554103949950999710565799465200849541325*cos(q2L))/1461501637330902918203684832716283019655932542976 - (329794241748012540206902858004467560228111939405*sin(q1L))/2993155353253689176481146537402947624255349848014848 - (67682029681889335677290557259385*cos(q2L)*((6283307137322267*cos(q1L))/9007199254740992 - (4872700232219253*sin(q1L))/9007199254740992))/332306998946228968225951765070086144 - (9007199067919185*sin(q2L)*((4872700232219253*cos(q1L))/9007199254740992 + (6283307137322267*sin(q1L))/9007199254740992))/9007199254740992 + 477861849958017465213997854626476001002268408317/24519928653854221733733552434404946937899825954937634816) + (7514214926474921*cos(q4L)*((9007199067919185*cos(q3L)*((56594998190739085871744456992395*cos(q1L))/81129638414606681695789005144064 - (43889380989894851923989405068805*sin(q1L))/81129638414606681695789005144064 + 63594381400292563045725890951477/664613997892457936451903530140172288))/9007199254740992 + (7514214926474921*cos(q3L)*((7514214926474921*cos(q2L)*((6283307137322267*cos(q1L))/9007199254740992 - (4872700232219253*sin(q1L))/9007199254740992))/36893488147419103232 - (76229820211215127867025072518845*cos(q2L))/162259276829213363391578010288128 + sin(q2L)*((4872700232219253*cos(q1L))/9007199254740992 + (6283307137322267*sin(q1L))/9007199254740992)))/36893488147419103232 - sin(q3L)*((76229820211215127867025072518845*sin(q2L))/162259276829213363391578010288128 + cos(q2L)*((4872700232219253*cos(q1L))/9007199254740992 + (6283307137322267*sin(q1L))/9007199254740992) - (7514214926474921*sin(q2L)*((6283307137322267*cos(q1L))/9007199254740992 - (4872700232219253*sin(q1L))/9007199254740992))/36893488147419103232)))/36893488147419103232))/36893488147419103232 - (9007199067919185*cos(q5L)*((666467732349846997487583938718911583194406904318712922873589125*cos(q1L))/113078212145816597093331040047546785012958969400039613319782796882727665664 + (1076049180065244948668759145796765391250102872519935285209856875*cos(q2L))/55213970774324510299478046898216203619608871777363092441300193790394368 - (516845254133432670685844229576986303733782399690601453662320875*sin(q1L))/113078212145816597093331040047546785012958969400039613319782796882727665664 - (81129635049124235038645691064225*cos(q3L)*((56594998190739085871744456992395*cos(q1L))/81129638414606681695789005144064 - (43889380989894851923989405068805*sin(q1L))/81129638414606681695789005144064 + 63594381400292563045725890951477/664613997892457936451903530140172288))/81129638414606681695789005144064 + (2115063383689692319117831580025*sin(q3L)*((56594998190739085871744456992395*cos(q1L))/81129638414606681695789005144064 - (43889380989894851923989405068805*sin(q1L))/81129638414606681695789005144064 + 63594381400292563045725890951477/664613997892457936451903530140172288))/10384593717069655257060992658440192 - (67682029681889335677290557259385*cos(q3L)*((7514214926474921*cos(q2L)*((6283307137322267*cos(q1L))/9007199254740992 - (4872700232219253*sin(q1L))/9007199254740992))/36893488147419103232 - (76229820211215127867025072518845*cos(q2L))/162259276829213363391578010288128 + sin(q2L)*((4872700232219253*cos(q1L))/9007199254740992 + (6283307137322267*sin(q1L))/9007199254740992)))/332306998946228968225951765070086144 + (234819211581865*cos(q3L)*((76229820211215127867025072518845*sin(q2L))/162259276829213363391578010288128 + cos(q2L)*((4872700232219253*cos(q1L))/9007199254740992 + (6283307137322267*sin(q1L))/9007199254740992) - (7514214926474921*sin(q2L)*((6283307137322267*cos(q1L))/9007199254740992 - (4872700232219253*sin(q1L))/9007199254740992))/36893488147419103232))/1152921504606846976 + (1764482024691522628700660907665*sin(q3L)*((7514214926474921*cos(q2L)*((6283307137322267*cos(q1L))/9007199254740992 - (4872700232219253*sin(q1L))/9007199254740992))/36893488147419103232 - (76229820211215127867025072518845*cos(q2L))/162259276829213363391578010288128 + sin(q2L)*((4872700232219253*cos(q1L))/9007199254740992 + (6283307137322267*sin(q1L))/9007199254740992)))/42535295865117307932921825928971026432 + (9007199067919185*sin(q3L)*((76229820211215127867025072518845*sin(q2L))/162259276829213363391578010288128 + cos(q2L)*((4872700232219253*cos(q1L))/9007199254740992 + (6283307137322267*sin(q1L))/9007199254740992) - (7514214926474921*sin(q2L)*((6283307137322267*cos(q1L))/9007199254740992 - (4872700232219253*sin(q1L))/9007199254740992))/36893488147419103232))/9007199254740992 - (106069577339469832923929692356850887620017617375*cos(q2L)*((6283307137322267*cos(q1L))/9007199254740992 - (4872700232219253*sin(q1L))/9007199254740992))/12554203470773361527671578846415332832204710888928069025792 - (14115856197532180673579726082375*sin(q2L)*((4872700232219253*cos(q1L))/9007199254740992 + (6283307137322267*sin(q1L))/9007199254740992))/340282366920938463463374607431768211456 + 748893091562634003789577347105888574211761174637088840996300475/926336713898529563388567880069503262826159877325124512315660672063305037119488))/9007199254740992 + sin(q5L)*(((7514214926474921*cos(q4L))/36893488147419103232 + (4503599440548691*sin(q4L))/4503599627370496)*((9007199067919185*sin(q3L)*((56594998190739085871744456992395*cos(q1L))/81129638414606681695789005144064 - (43889380989894851923989405068805*sin(q1L))/81129638414606681695789005144064 + 63594381400292563045725890951477/664613997892457936451903530140172288))/9007199254740992 + cos(q3L)*((76229820211215127867025072518845*sin(q2L))/162259276829213363391578010288128 + cos(q2L)*((4872700232219253*cos(q1L))/9007199254740992 + (6283307137322267*sin(q1L))/9007199254740992) - (7514214926474921*sin(q2L)*((6283307137322267*cos(q1L))/9007199254740992 - (4872700232219253*sin(q1L))/9007199254740992))/36893488147419103232) + (7514214926474921*sin(q3L)*((7514214926474921*cos(q2L)*((6283307137322267*cos(q1L))/9007199254740992 - (4872700232219253*sin(q1L))/9007199254740992))/36893488147419103232 - (76229820211215127867025072518845*cos(q2L))/162259276829213363391578010288128 + sin(q2L)*((4872700232219253*cos(q1L))/9007199254740992 + (6283307137322267*sin(q1L))/9007199254740992)))/36893488147419103232) - ((9007199067919185*cos(q4L))/9007199254740992 - (234819211581865*sin(q4L))/1152921504606846976)*((425266980168672787164801917791314326747055225795*cos(q1L))/2993155353253689176481146537402947624255349848014848 + (686617165554103949950999710565799465200849541325*cos(q2L))/1461501637330902918203684832716283019655932542976 - (329794241748012540206902858004467560228111939405*sin(q1L))/2993155353253689176481146537402947624255349848014848 - (67682029681889335677290557259385*cos(q2L)*((6283307137322267*cos(q1L))/9007199254740992 - (4872700232219253*sin(q1L))/9007199254740992))/332306998946228968225951765070086144 - (9007199067919185*sin(q2L)*((4872700232219253*cos(q1L))/9007199254740992 + (6283307137322267*sin(q1L))/9007199254740992))/9007199254740992 + 477861849958017465213997854626476001002268408317/24519928653854221733733552434404946937899825954937634816) + (7514214926474921*sin(q4L)*((9007199067919185*cos(q3L)*((56594998190739085871744456992395*cos(q1L))/81129638414606681695789005144064 - (43889380989894851923989405068805*sin(q1L))/81129638414606681695789005144064 + 63594381400292563045725890951477/664613997892457936451903530140172288))/9007199254740992 + (7514214926474921*cos(q3L)*((7514214926474921*cos(q2L)*((6283307137322267*cos(q1L))/9007199254740992 - (4872700232219253*sin(q1L))/9007199254740992))/36893488147419103232 - (76229820211215127867025072518845*cos(q2L))/162259276829213363391578010288128 + sin(q2L)*((4872700232219253*cos(q1L))/9007199254740992 + (6283307137322267*sin(q1L))/9007199254740992)))/36893488147419103232 - sin(q3L)*((76229820211215127867025072518845*sin(q2L))/162259276829213363391578010288128 + cos(q2L)*((4872700232219253*cos(q1L))/9007199254740992 + (6283307137322267*sin(q1L))/9007199254740992) - (7514214926474921*sin(q2L)*((6283307137322267*cos(q1L))/9007199254740992 - (4872700232219253*sin(q1L))/9007199254740992))/36893488147419103232)))/36893488147419103232)))/9007199254740992000 - (202883803014822867*sin(q6L)*((9007199067919185*sin(q5L)*((666467732349846997487583938718911583194406904318712922873589125*cos(q1L))/113078212145816597093331040047546785012958969400039613319782796882727665664 + (1076049180065244948668759145796765391250102872519935285209856875*cos(q2L))/55213970774324510299478046898216203619608871777363092441300193790394368 - (516845254133432670685844229576986303733782399690601453662320875*sin(q1L))/113078212145816597093331040047546785012958969400039613319782796882727665664 - (81129635049124235038645691064225*cos(q3L)*((56594998190739085871744456992395*cos(q1L))/81129638414606681695789005144064 - (43889380989894851923989405068805*sin(q1L))/81129638414606681695789005144064 + 63594381400292563045725890951477/664613997892457936451903530140172288))/81129638414606681695789005144064 + (2115063383689692319117831580025*sin(q3L)*((56594998190739085871744456992395*cos(q1L))/81129638414606681695789005144064 - (43889380989894851923989405068805*sin(q1L))/81129638414606681695789005144064 + 63594381400292563045725890951477/664613997892457936451903530140172288))/10384593717069655257060992658440192 - (67682029681889335677290557259385*cos(q3L)*((7514214926474921*cos(q2L)*((6283307137322267*cos(q1L))/9007199254740992 - (4872700232219253*sin(q1L))/9007199254740992))/36893488147419103232 - (76229820211215127867025072518845*cos(q2L))/162259276829213363391578010288128 + sin(q2L)*((4872700232219253*cos(q1L))/9007199254740992 + (6283307137322267*sin(q1L))/9007199254740992)))/332306998946228968225951765070086144 + (234819211581865*cos(q3L)*((76229820211215127867025072518845*sin(q2L))/162259276829213363391578010288128 + cos(q2L)*((4872700232219253*cos(q1L))/9007199254740992 + (6283307137322267*sin(q1L))/9007199254740992) - (7514214926474921*sin(q2L)*((6283307137322267*cos(q1L))/9007199254740992 - (4872700232219253*sin(q1L))/9007199254740992))/36893488147419103232))/1152921504606846976 + (1764482024691522628700660907665*sin(q3L)*((7514214926474921*cos(q2L)*((6283307137322267*cos(q1L))/9007199254740992 - (4872700232219253*sin(q1L))/9007199254740992))/36893488147419103232 - (76229820211215127867025072518845*cos(q2L))/162259276829213363391578010288128 + sin(q2L)*((4872700232219253*cos(q1L))/9007199254740992 + (6283307137322267*sin(q1L))/9007199254740992)))/42535295865117307932921825928971026432 + (9007199067919185*sin(q3L)*((76229820211215127867025072518845*sin(q2L))/162259276829213363391578010288128 + cos(q2L)*((4872700232219253*cos(q1L))/9007199254740992 + (6283307137322267*sin(q1L))/9007199254740992) - (7514214926474921*sin(q2L)*((6283307137322267*cos(q1L))/9007199254740992 - (4872700232219253*sin(q1L))/9007199254740992))/36893488147419103232))/9007199254740992 - (106069577339469832923929692356850887620017617375*cos(q2L)*((6283307137322267*cos(q1L))/9007199254740992 - (4872700232219253*sin(q1L))/9007199254740992))/12554203470773361527671578846415332832204710888928069025792 - (14115856197532180673579726082375*sin(q2L)*((4872700232219253*cos(q1L))/9007199254740992 + (6283307137322267*sin(q1L))/9007199254740992))/340282366920938463463374607431768211456 + 748893091562634003789577347105888574211761174637088840996300475/926336713898529563388567880069503262826159877325124512315660672063305037119488))/9007199254740992 - (7514214926474921*sin(q5L)*(((4503599440548691*cos(q4L))/4503599627370496 - (7514214926474921*sin(q4L))/36893488147419103232)*((9007199067919185*sin(q3L)*((56594998190739085871744456992395*cos(q1L))/81129638414606681695789005144064 - (43889380989894851923989405068805*sin(q1L))/81129638414606681695789005144064 + 63594381400292563045725890951477/664613997892457936451903530140172288))/9007199254740992 + cos(q3L)*((76229820211215127867025072518845*sin(q2L))/162259276829213363391578010288128 + cos(q2L)*((4872700232219253*cos(q1L))/9007199254740992 + (6283307137322267*sin(q1L))/9007199254740992) - (7514214926474921*sin(q2L)*((6283307137322267*cos(q1L))/9007199254740992 - (4872700232219253*sin(q1L))/9007199254740992))/36893488147419103232) + (7514214926474921*sin(q3L)*((7514214926474921*cos(q2L)*((6283307137322267*cos(q1L))/9007199254740992 - (4872700232219253*sin(q1L))/9007199254740992))/36893488147419103232 - (76229820211215127867025072518845*cos(q2L))/162259276829213363391578010288128 + sin(q2L)*((4872700232219253*cos(q1L))/9007199254740992 + (6283307137322267*sin(q1L))/9007199254740992)))/36893488147419103232) + ((234819211581865*cos(q4L))/1152921504606846976 + (9007199067919185*sin(q4L))/9007199254740992)*((425266980168672787164801917791314326747055225795*cos(q1L))/2993155353253689176481146537402947624255349848014848 + (686617165554103949950999710565799465200849541325*cos(q2L))/1461501637330902918203684832716283019655932542976 - (329794241748012540206902858004467560228111939405*sin(q1L))/2993155353253689176481146537402947624255349848014848 - (67682029681889335677290557259385*cos(q2L)*((6283307137322267*cos(q1L))/9007199254740992 - (4872700232219253*sin(q1L))/9007199254740992))/332306998946228968225951765070086144 - (9007199067919185*sin(q2L)*((4872700232219253*cos(q1L))/9007199254740992 + (6283307137322267*sin(q1L))/9007199254740992))/9007199254740992 + 477861849958017465213997854626476001002268408317/24519928653854221733733552434404946937899825954937634816) + (7514214926474921*cos(q4L)*((9007199067919185*cos(q3L)*((56594998190739085871744456992395*cos(q1L))/81129638414606681695789005144064 - (43889380989894851923989405068805*sin(q1L))/81129638414606681695789005144064 + 63594381400292563045725890951477/664613997892457936451903530140172288))/9007199254740992 + (7514214926474921*cos(q3L)*((7514214926474921*cos(q2L)*((6283307137322267*cos(q1L))/9007199254740992 - (4872700232219253*sin(q1L))/9007199254740992))/36893488147419103232 - (76229820211215127867025072518845*cos(q2L))/162259276829213363391578010288128 + sin(q2L)*((4872700232219253*cos(q1L))/9007199254740992 + (6283307137322267*sin(q1L))/9007199254740992)))/36893488147419103232 - sin(q3L)*((76229820211215127867025072518845*sin(q2L))/162259276829213363391578010288128 + cos(q2L)*((4872700232219253*cos(q1L))/9007199254740992 + (6283307137322267*sin(q1L))/9007199254740992) - (7514214926474921*sin(q2L)*((6283307137322267*cos(q1L))/9007199254740992 - (4872700232219253*sin(q1L))/9007199254740992))/36893488147419103232)))/36893488147419103232))/36893488147419103232 + cos(q5L)*(((7514214926474921*cos(q4L))/36893488147419103232 + (4503599440548691*sin(q4L))/4503599627370496)*((9007199067919185*sin(q3L)*((56594998190739085871744456992395*cos(q1L))/81129638414606681695789005144064 - (43889380989894851923989405068805*sin(q1L))/81129638414606681695789005144064 + 63594381400292563045725890951477/664613997892457936451903530140172288))/9007199254740992 + cos(q3L)*((76229820211215127867025072518845*sin(q2L))/162259276829213363391578010288128 + cos(q2L)*((4872700232219253*cos(q1L))/9007199254740992 + (6283307137322267*sin(q1L))/9007199254740992) - (7514214926474921*sin(q2L)*((6283307137322267*cos(q1L))/9007199254740992 - (4872700232219253*sin(q1L))/9007199254740992))/36893488147419103232) + (7514214926474921*sin(q3L)*((7514214926474921*cos(q2L)*((6283307137322267*cos(q1L))/9007199254740992 - (4872700232219253*sin(q1L))/9007199254740992))/36893488147419103232 - (76229820211215127867025072518845*cos(q2L))/162259276829213363391578010288128 + sin(q2L)*((4872700232219253*cos(q1L))/9007199254740992 + (6283307137322267*sin(q1L))/9007199254740992)))/36893488147419103232) - ((9007199067919185*cos(q4L))/9007199254740992 - (234819211581865*sin(q4L))/1152921504606846976)*((425266980168672787164801917791314326747055225795*cos(q1L))/2993155353253689176481146537402947624255349848014848 + (686617165554103949950999710565799465200849541325*cos(q2L))/1461501637330902918203684832716283019655932542976 - (329794241748012540206902858004467560228111939405*sin(q1L))/2993155353253689176481146537402947624255349848014848 - (67682029681889335677290557259385*cos(q2L)*((6283307137322267*cos(q1L))/9007199254740992 - (4872700232219253*sin(q1L))/9007199254740992))/332306998946228968225951765070086144 - (9007199067919185*sin(q2L)*((4872700232219253*cos(q1L))/9007199254740992 + (6283307137322267*sin(q1L))/9007199254740992))/9007199254740992 + 477861849958017465213997854626476001002268408317/24519928653854221733733552434404946937899825954937634816) + (7514214926474921*sin(q4L)*((9007199067919185*cos(q3L)*((56594998190739085871744456992395*cos(q1L))/81129638414606681695789005144064 - (43889380989894851923989405068805*sin(q1L))/81129638414606681695789005144064 + 63594381400292563045725890951477/664613997892457936451903530140172288))/9007199254740992 + (7514214926474921*cos(q3L)*((7514214926474921*cos(q2L)*((6283307137322267*cos(q1L))/9007199254740992 - (4872700232219253*sin(q1L))/9007199254740992))/36893488147419103232 - (76229820211215127867025072518845*cos(q2L))/162259276829213363391578010288128 + sin(q2L)*((4872700232219253*cos(q1L))/9007199254740992 + (6283307137322267*sin(q1L))/9007199254740992)))/36893488147419103232 - sin(q3L)*((76229820211215127867025072518845*sin(q2L))/162259276829213363391578010288128 + cos(q2L)*((4872700232219253*cos(q1L))/9007199254740992 + (6283307137322267*sin(q1L))/9007199254740992) - (7514214926474921*sin(q2L)*((6283307137322267*cos(q1L))/9007199254740992 - (4872700232219253*sin(q1L))/9007199254740992))/36893488147419103232)))/36893488147419103232)))/36893488147419103232000, (584133382113593486367040631332731*sin(q6L)*((5007981782437112884252809417893315588674027328151397427571757674310327570834125*cos(q1L))/4171849679533027504677776769862406473833407270227837441302815640277772901915313574263597826048 + (8085664810467363599778659999511780427732698420102663058998013758035866686931875*cos(q2L))/2037035976334486086268445688409378161051468393665936250636140449354381299763336706183397376 - (3883686323287163634621917344193152976968889150546766896070169015701143342275875*sin(q1L))/4171849679533027504677776769862406473833407270227837441302815640277772901915313574263597826048 - (609625514665592237562888769449172969868262801225*cos(q3L)*((56594998190739085871744456992395*cos(q1L))/81129638414606681695789005144064 - (43889380989894851923989405068805*sin(q1L))/81129638414606681695789005144064 + 63594381400292563045725890951477/664613997892457936451903530140172288))/2993155353253689176481146537402947624255349848014848 + (15893040848161638993908057577265778144967053025*sin(q3L)*((56594998190739085871744456992395*cos(q1L))/81129638414606681695789005144064 - (43889380989894851923989405068805*sin(q1L))/81129638414606681695789005144064 + 63594381400292563045725890951477/664613997892457936451903530140172288))/383123885216472214589586756787577295904684780545900544 + (9007199067919185*((4503599440548691*cos(q4L))/4503599627370496 - (7514214926474921*sin(q4L))/36893488147419103232)*((9007199067919185*sin(q3L)*((56594998190739085871744456992395*cos(q1L))/81129638414606681695789005144064 - (43889380989894851923989405068805*sin(q1L))/81129638414606681695789005144064 + 63594381400292563045725890951477/664613997892457936451903530140172288))/9007199254740992 + cos(q3L)*((76229820211215127867025072518845*sin(q2L))/162259276829213363391578010288128 + cos(q2L)*((4872700232219253*cos(q1L))/9007199254740992 + (6283307137322267*sin(q1L))/9007199254740992) - (7514214926474921*sin(q2L)*((6283307137322267*cos(q1L))/9007199254740992 - (4872700232219253*sin(q1L))/9007199254740992))/36893488147419103232) + (7514214926474921*sin(q3L)*((7514214926474921*cos(q2L)*((6283307137322267*cos(q1L))/9007199254740992 - (4872700232219253*sin(q1L))/9007199254740992))/36893488147419103232 - (76229820211215127867025072518845*cos(q2L))/162259276829213363391578010288128 + sin(q2L)*((4872700232219253*cos(q1L))/9007199254740992 + (6283307137322267*sin(q1L))/9007199254740992)))/36893488147419103232))/9007199254740992 + (9007199067919185*((234819211581865*cos(q4L))/1152921504606846976 + (9007199067919185*sin(q4L))/9007199254740992)*((425266980168672787164801917791314326747055225795*cos(q1L))/2993155353253689176481146537402947624255349848014848 + (686617165554103949950999710565799465200849541325*cos(q2L))/1461501637330902918203684832716283019655932542976 - (329794241748012540206902858004467560228111939405*sin(q1L))/2993155353253689176481146537402947624255349848014848 - (67682029681889335677290557259385*cos(q2L)*((6283307137322267*cos(q1L))/9007199254740992 - (4872700232219253*sin(q1L))/9007199254740992))/332306998946228968225951765070086144 - (9007199067919185*sin(q2L)*((4872700232219253*cos(q1L))/9007199254740992 + (6283307137322267*sin(q1L))/9007199254740992))/9007199254740992 + 477861849958017465213997854626476001002268408317/24519928653854221733733552434404946937899825954937634816))/9007199254740992 - (508577317689771495245073589786522929324694383585*cos(q3L)*((7514214926474921*cos(q2L)*((6283307137322267*cos(q1L))/9007199254740992 - (4872700232219253*sin(q1L))/9007199254740992))/36893488147419103232 - (76229820211215127867025072518845*cos(q2L))/162259276829213363391578010288128 + sin(q2L)*((4872700232219253*cos(q1L))/9007199254740992 + (6283307137322267*sin(q1L))/9007199254740992)))/12259964326927110866866776217202473468949912977468817408 + (1764482024691522628700660907665*cos(q3L)*((76229820211215127867025072518845*sin(q2L))/162259276829213363391578010288128 + cos(q2L)*((4872700232219253*cos(q1L))/9007199254740992 + (6283307137322267*sin(q1L))/9007199254740992) - (7514214926474921*sin(q2L)*((6283307137322267*cos(q1L))/9007199254740992 - (4872700232219253*sin(q1L))/9007199254740992))/36893488147419103232))/42535295865117307932921825928971026432 + (13258697167433729449897784796786197386719169465*sin(q3L)*((7514214926474921*cos(q2L)*((6283307137322267*cos(q1L))/9007199254740992 - (4872700232219253*sin(q1L))/9007199254740992))/36893488147419103232 - (76229820211215127867025072518845*cos(q2L))/162259276829213363391578010288128 + sin(q2L)*((4872700232219253*cos(q1L))/9007199254740992 + (6283307137322267*sin(q1L))/9007199254740992)))/1569275433846670190958947355801916604025588861116008628224 + (67682029681889335677290557259385*sin(q3L)*((76229820211215127867025072518845*sin(q2L))/162259276829213363391578010288128 + cos(q2L)*((4872700232219253*cos(q1L))/9007199254740992 + (6283307137322267*sin(q1L))/9007199254740992) - (7514214926474921*sin(q2L)*((6283307137322267*cos(q1L))/9007199254740992 - (4872700232219253*sin(q1L))/9007199254740992))/36893488147419103232))/332306998946228968225951765070086144 - (797029601289130257223357069404502671534492977261568326111352375*cos(q2L)*((6283307137322267*cos(q1L))/9007199254740992 - (4872700232219253*sin(q1L))/9007199254740992))/463168356949264781694283940034751631413079938662562256157830336031652518559744 - (106069577339469832923929692356850887620017617375*sin(q2L)*((4872700232219253*cos(q1L))/9007199254740992 + (6283307137322267*sin(q1L))/9007199254740992))/12554203470773361527671578846415332832204710888928069025792 + (67682029681889335677290557259385*cos(q4L)*((9007199067919185*cos(q3L)*((56594998190739085871744456992395*cos(q1L))/81129638414606681695789005144064 - (43889380989894851923989405068805*sin(q1L))/81129638414606681695789005144064 + 63594381400292563045725890951477/664613997892457936451903530140172288))/9007199254740992 + (7514214926474921*cos(q3L)*((7514214926474921*cos(q2L)*((6283307137322267*cos(q1L))/9007199254740992 - (4872700232219253*sin(q1L))/9007199254740992))/36893488147419103232 - (76229820211215127867025072518845*cos(q2L))/162259276829213363391578010288128 + sin(q2L)*((4872700232219253*cos(q1L))/9007199254740992 + (6283307137322267*sin(q1L))/9007199254740992)))/36893488147419103232 - sin(q3L)*((76229820211215127867025072518845*sin(q2L))/162259276829213363391578010288128 + cos(q2L)*((4872700232219253*cos(q1L))/9007199254740992 + (6283307137322267*sin(q1L))/9007199254740992) - (7514214926474921*sin(q2L)*((6283307137322267*cos(q1L))/9007199254740992 - (4872700232219253*sin(q1L))/9007199254740992))/36893488147419103232)))/332306998946228968225951765070086144 + 5627343646953894151088800368568300690099750210758529431022262609480693867887475/34175792574734561318320347298712833833643272357706444319152665725155515612490248800367393390985216))/16225927682921336339157801028812800 - (48638874966763599*cos(q6L)*((5007981782437112884252809417893315588674027328151397427571757674310327570834125*cos(q1L))/4171849679533027504677776769862406473833407270227837441302815640277772901915313574263597826048 + (8085664810467363599778659999511780427732698420102663058998013758035866686931875*cos(q2L))/2037035976334486086268445688409378161051468393665936250636140449354381299763336706183397376 - (3883686323287163634621917344193152976968889150546766896070169015701143342275875*sin(q1L))/4171849679533027504677776769862406473833407270227837441302815640277772901915313574263597826048 - (609625514665592237562888769449172969868262801225*cos(q3L)*((56594998190739085871744456992395*cos(q1L))/81129638414606681695789005144064 - (43889380989894851923989405068805*sin(q1L))/81129638414606681695789005144064 + 63594381400292563045725890951477/664613997892457936451903530140172288))/2993155353253689176481146537402947624255349848014848 + (15893040848161638993908057577265778144967053025*sin(q3L)*((56594998190739085871744456992395*cos(q1L))/81129638414606681695789005144064 - (43889380989894851923989405068805*sin(q1L))/81129638414606681695789005144064 + 63594381400292563045725890951477/664613997892457936451903530140172288))/383123885216472214589586756787577295904684780545900544 + (9007199067919185*((4503599440548691*cos(q4L))/4503599627370496 - (7514214926474921*sin(q4L))/36893488147419103232)*((9007199067919185*sin(q3L)*((56594998190739085871744456992395*cos(q1L))/81129638414606681695789005144064 - (43889380989894851923989405068805*sin(q1L))/81129638414606681695789005144064 + 63594381400292563045725890951477/664613997892457936451903530140172288))/9007199254740992 + cos(q3L)*((76229820211215127867025072518845*sin(q2L))/162259276829213363391578010288128 + cos(q2L)*((4872700232219253*cos(q1L))/9007199254740992 + (6283307137322267*sin(q1L))/9007199254740992) - (7514214926474921*sin(q2L)*((6283307137322267*cos(q1L))/9007199254740992 - (4872700232219253*sin(q1L))/9007199254740992))/36893488147419103232) + (7514214926474921*sin(q3L)*((7514214926474921*cos(q2L)*((6283307137322267*cos(q1L))/9007199254740992 - (4872700232219253*sin(q1L))/9007199254740992))/36893488147419103232 - (76229820211215127867025072518845*cos(q2L))/162259276829213363391578010288128 + sin(q2L)*((4872700232219253*cos(q1L))/9007199254740992 + (6283307137322267*sin(q1L))/9007199254740992)))/36893488147419103232))/9007199254740992 + (9007199067919185*((234819211581865*cos(q4L))/1152921504606846976 + (9007199067919185*sin(q4L))/9007199254740992)*((425266980168672787164801917791314326747055225795*cos(q1L))/2993155353253689176481146537402947624255349848014848 + (686617165554103949950999710565799465200849541325*cos(q2L))/1461501637330902918203684832716283019655932542976 - (329794241748012540206902858004467560228111939405*sin(q1L))/2993155353253689176481146537402947624255349848014848 - (67682029681889335677290557259385*cos(q2L)*((6283307137322267*cos(q1L))/9007199254740992 - (4872700232219253*sin(q1L))/9007199254740992))/332306998946228968225951765070086144 - (9007199067919185*sin(q2L)*((4872700232219253*cos(q1L))/9007199254740992 + (6283307137322267*sin(q1L))/9007199254740992))/9007199254740992 + 477861849958017465213997854626476001002268408317/24519928653854221733733552434404946937899825954937634816))/9007199254740992 - (508577317689771495245073589786522929324694383585*cos(q3L)*((7514214926474921*cos(q2L)*((6283307137322267*cos(q1L))/9007199254740992 - (4872700232219253*sin(q1L))/9007199254740992))/36893488147419103232 - (76229820211215127867025072518845*cos(q2L))/162259276829213363391578010288128 + sin(q2L)*((4872700232219253*cos(q1L))/9007199254740992 + (6283307137322267*sin(q1L))/9007199254740992)))/12259964326927110866866776217202473468949912977468817408 + (1764482024691522628700660907665*cos(q3L)*((76229820211215127867025072518845*sin(q2L))/162259276829213363391578010288128 + cos(q2L)*((4872700232219253*cos(q1L))/9007199254740992 + (6283307137322267*sin(q1L))/9007199254740992) - (7514214926474921*sin(q2L)*((6283307137322267*cos(q1L))/9007199254740992 - (4872700232219253*sin(q1L))/9007199254740992))/36893488147419103232))/42535295865117307932921825928971026432 + (13258697167433729449897784796786197386719169465*sin(q3L)*((7514214926474921*cos(q2L)*((6283307137322267*cos(q1L))/9007199254740992 - (4872700232219253*sin(q1L))/9007199254740992))/36893488147419103232 - (76229820211215127867025072518845*cos(q2L))/162259276829213363391578010288128 + sin(q2L)*((4872700232219253*cos(q1L))/9007199254740992 + (6283307137322267*sin(q1L))/9007199254740992)))/1569275433846670190958947355801916604025588861116008628224 + (67682029681889335677290557259385*sin(q3L)*((76229820211215127867025072518845*sin(q2L))/162259276829213363391578010288128 + cos(q2L)*((4872700232219253*cos(q1L))/9007199254740992 + (6283307137322267*sin(q1L))/9007199254740992) - (7514214926474921*sin(q2L)*((6283307137322267*cos(q1L))/9007199254740992 - (4872700232219253*sin(q1L))/9007199254740992))/36893488147419103232))/332306998946228968225951765070086144 - (797029601289130257223357069404502671534492977261568326111352375*cos(q2L)*((6283307137322267*cos(q1L))/9007199254740992 - (4872700232219253*sin(q1L))/9007199254740992))/463168356949264781694283940034751631413079938662562256157830336031652518559744 - (106069577339469832923929692356850887620017617375*sin(q2L)*((4872700232219253*cos(q1L))/9007199254740992 + (6283307137322267*sin(q1L))/9007199254740992))/12554203470773361527671578846415332832204710888928069025792 + (67682029681889335677290557259385*cos(q4L)*((9007199067919185*cos(q3L)*((56594998190739085871744456992395*cos(q1L))/81129638414606681695789005144064 - (43889380989894851923989405068805*sin(q1L))/81129638414606681695789005144064 + 63594381400292563045725890951477/664613997892457936451903530140172288))/9007199254740992 + (7514214926474921*cos(q3L)*((7514214926474921*cos(q2L)*((6283307137322267*cos(q1L))/9007199254740992 - (4872700232219253*sin(q1L))/9007199254740992))/36893488147419103232 - (76229820211215127867025072518845*cos(q2L))/162259276829213363391578010288128 + sin(q2L)*((4872700232219253*cos(q1L))/9007199254740992 + (6283307137322267*sin(q1L))/9007199254740992)))/36893488147419103232 - sin(q3L)*((76229820211215127867025072518845*sin(q2L))/162259276829213363391578010288128 + cos(q2L)*((4872700232219253*cos(q1L))/9007199254740992 + (6283307137322267*sin(q1L))/9007199254740992) - (7514214926474921*sin(q2L)*((6283307137322267*cos(q1L))/9007199254740992 - (4872700232219253*sin(q1L))/9007199254740992))/36893488147419103232)))/332306998946228968225951765070086144 + 5627343646953894151088800368568300690099750210758529431022262609480693867887475/34175792574734561318320347298712833833643272357706444319152665725155515612490248800367393390985216))/1801439850948198400 - (202883803014822867*cos(q6L)*((7514214926474921*cos(q5L)*(((4503599440548691*cos(q4L))/4503599627370496 - (7514214926474921*sin(q4L))/36893488147419103232)*((9007199067919185*sin(q3L)*((56594998190739085871744456992395*cos(q1L))/81129638414606681695789005144064 - (43889380989894851923989405068805*sin(q1L))/81129638414606681695789005144064 + 63594381400292563045725890951477/664613997892457936451903530140172288))/9007199254740992 + cos(q3L)*((76229820211215127867025072518845*sin(q2L))/162259276829213363391578010288128 + cos(q2L)*((4872700232219253*cos(q1L))/9007199254740992 + (6283307137322267*sin(q1L))/9007199254740992) - (7514214926474921*sin(q2L)*((6283307137322267*cos(q1L))/9007199254740992 - (4872700232219253*sin(q1L))/9007199254740992))/36893488147419103232) + (7514214926474921*sin(q3L)*((7514214926474921*cos(q2L)*((6283307137322267*cos(q1L))/9007199254740992 - (4872700232219253*sin(q1L))/9007199254740992))/36893488147419103232 - (76229820211215127867025072518845*cos(q2L))/162259276829213363391578010288128 + sin(q2L)*((4872700232219253*cos(q1L))/9007199254740992 + (6283307137322267*sin(q1L))/9007199254740992)))/36893488147419103232) + ((234819211581865*cos(q4L))/1152921504606846976 + (9007199067919185*sin(q4L))/9007199254740992)*((425266980168672787164801917791314326747055225795*cos(q1L))/2993155353253689176481146537402947624255349848014848 + (686617165554103949950999710565799465200849541325*cos(q2L))/1461501637330902918203684832716283019655932542976 - (329794241748012540206902858004467560228111939405*sin(q1L))/2993155353253689176481146537402947624255349848014848 - (67682029681889335677290557259385*cos(q2L)*((6283307137322267*cos(q1L))/9007199254740992 - (4872700232219253*sin(q1L))/9007199254740992))/332306998946228968225951765070086144 - (9007199067919185*sin(q2L)*((4872700232219253*cos(q1L))/9007199254740992 + (6283307137322267*sin(q1L))/9007199254740992))/9007199254740992 + 477861849958017465213997854626476001002268408317/24519928653854221733733552434404946937899825954937634816) + (7514214926474921*cos(q4L)*((9007199067919185*cos(q3L)*((56594998190739085871744456992395*cos(q1L))/81129638414606681695789005144064 - (43889380989894851923989405068805*sin(q1L))/81129638414606681695789005144064 + 63594381400292563045725890951477/664613997892457936451903530140172288))/9007199254740992 + (7514214926474921*cos(q3L)*((7514214926474921*cos(q2L)*((6283307137322267*cos(q1L))/9007199254740992 - (4872700232219253*sin(q1L))/9007199254740992))/36893488147419103232 - (76229820211215127867025072518845*cos(q2L))/162259276829213363391578010288128 + sin(q2L)*((4872700232219253*cos(q1L))/9007199254740992 + (6283307137322267*sin(q1L))/9007199254740992)))/36893488147419103232 - sin(q3L)*((76229820211215127867025072518845*sin(q2L))/162259276829213363391578010288128 + cos(q2L)*((4872700232219253*cos(q1L))/9007199254740992 + (6283307137322267*sin(q1L))/9007199254740992) - (7514214926474921*sin(q2L)*((6283307137322267*cos(q1L))/9007199254740992 - (4872700232219253*sin(q1L))/9007199254740992))/36893488147419103232)))/36893488147419103232))/36893488147419103232 - (9007199067919185*cos(q5L)*((666467732349846997487583938718911583194406904318712922873589125*cos(q1L))/113078212145816597093331040047546785012958969400039613319782796882727665664 + (1076049180065244948668759145796765391250102872519935285209856875*cos(q2L))/55213970774324510299478046898216203619608871777363092441300193790394368 - (516845254133432670685844229576986303733782399690601453662320875*sin(q1L))/113078212145816597093331040047546785012958969400039613319782796882727665664 - (81129635049124235038645691064225*cos(q3L)*((56594998190739085871744456992395*cos(q1L))/81129638414606681695789005144064 - (43889380989894851923989405068805*sin(q1L))/81129638414606681695789005144064 + 63594381400292563045725890951477/664613997892457936451903530140172288))/81129638414606681695789005144064 + (2115063383689692319117831580025*sin(q3L)*((56594998190739085871744456992395*cos(q1L))/81129638414606681695789005144064 - (43889380989894851923989405068805*sin(q1L))/81129638414606681695789005144064 + 63594381400292563045725890951477/664613997892457936451903530140172288))/10384593717069655257060992658440192 - (67682029681889335677290557259385*cos(q3L)*((7514214926474921*cos(q2L)*((6283307137322267*cos(q1L))/9007199254740992 - (4872700232219253*sin(q1L))/9007199254740992))/36893488147419103232 - (76229820211215127867025072518845*cos(q2L))/162259276829213363391578010288128 + sin(q2L)*((4872700232219253*cos(q1L))/9007199254740992 + (6283307137322267*sin(q1L))/9007199254740992)))/332306998946228968225951765070086144 + (234819211581865*cos(q3L)*((76229820211215127867025072518845*sin(q2L))/162259276829213363391578010288128 + cos(q2L)*((4872700232219253*cos(q1L))/9007199254740992 + (6283307137322267*sin(q1L))/9007199254740992) - (7514214926474921*sin(q2L)*((6283307137322267*cos(q1L))/9007199254740992 - (4872700232219253*sin(q1L))/9007199254740992))/36893488147419103232))/1152921504606846976 + (1764482024691522628700660907665*sin(q3L)*((7514214926474921*cos(q2L)*((6283307137322267*cos(q1L))/9007199254740992 - (4872700232219253*sin(q1L))/9007199254740992))/36893488147419103232 - (76229820211215127867025072518845*cos(q2L))/162259276829213363391578010288128 + sin(q2L)*((4872700232219253*cos(q1L))/9007199254740992 + (6283307137322267*sin(q1L))/9007199254740992)))/42535295865117307932921825928971026432 + (9007199067919185*sin(q3L)*((76229820211215127867025072518845*sin(q2L))/162259276829213363391578010288128 + cos(q2L)*((4872700232219253*cos(q1L))/9007199254740992 + (6283307137322267*sin(q1L))/9007199254740992) - (7514214926474921*sin(q2L)*((6283307137322267*cos(q1L))/9007199254740992 - (4872700232219253*sin(q1L))/9007199254740992))/36893488147419103232))/9007199254740992 - (106069577339469832923929692356850887620017617375*cos(q2L)*((6283307137322267*cos(q1L))/9007199254740992 - (4872700232219253*sin(q1L))/9007199254740992))/12554203470773361527671578846415332832204710888928069025792 - (14115856197532180673579726082375*sin(q2L)*((4872700232219253*cos(q1L))/9007199254740992 + (6283307137322267*sin(q1L))/9007199254740992))/340282366920938463463374607431768211456 + 748893091562634003789577347105888574211761174637088840996300475/926336713898529563388567880069503262826159877325124512315660672063305037119488))/9007199254740992 + sin(q5L)*(((7514214926474921*cos(q4L))/36893488147419103232 + (4503599440548691*sin(q4L))/4503599627370496)*((9007199067919185*sin(q3L)*((56594998190739085871744456992395*cos(q1L))/81129638414606681695789005144064 - (43889380989894851923989405068805*sin(q1L))/81129638414606681695789005144064 + 63594381400292563045725890951477/664613997892457936451903530140172288))/9007199254740992 + cos(q3L)*((76229820211215127867025072518845*sin(q2L))/162259276829213363391578010288128 + cos(q2L)*((4872700232219253*cos(q1L))/9007199254740992 + (6283307137322267*sin(q1L))/9007199254740992) - (7514214926474921*sin(q2L)*((6283307137322267*cos(q1L))/9007199254740992 - (4872700232219253*sin(q1L))/9007199254740992))/36893488147419103232) + (7514214926474921*sin(q3L)*((7514214926474921*cos(q2L)*((6283307137322267*cos(q1L))/9007199254740992 - (4872700232219253*sin(q1L))/9007199254740992))/36893488147419103232 - (76229820211215127867025072518845*cos(q2L))/162259276829213363391578010288128 + sin(q2L)*((4872700232219253*cos(q1L))/9007199254740992 + (6283307137322267*sin(q1L))/9007199254740992)))/36893488147419103232) - ((9007199067919185*cos(q4L))/9007199254740992 - (234819211581865*sin(q4L))/1152921504606846976)*((425266980168672787164801917791314326747055225795*cos(q1L))/2993155353253689176481146537402947624255349848014848 + (686617165554103949950999710565799465200849541325*cos(q2L))/1461501637330902918203684832716283019655932542976 - (329794241748012540206902858004467560228111939405*sin(q1L))/2993155353253689176481146537402947624255349848014848 - (67682029681889335677290557259385*cos(q2L)*((6283307137322267*cos(q1L))/9007199254740992 - (4872700232219253*sin(q1L))/9007199254740992))/332306998946228968225951765070086144 - (9007199067919185*sin(q2L)*((4872700232219253*cos(q1L))/9007199254740992 + (6283307137322267*sin(q1L))/9007199254740992))/9007199254740992 + 477861849958017465213997854626476001002268408317/24519928653854221733733552434404946937899825954937634816) + (7514214926474921*sin(q4L)*((9007199067919185*cos(q3L)*((56594998190739085871744456992395*cos(q1L))/81129638414606681695789005144064 - (43889380989894851923989405068805*sin(q1L))/81129638414606681695789005144064 + 63594381400292563045725890951477/664613997892457936451903530140172288))/9007199254740992 + (7514214926474921*cos(q3L)*((7514214926474921*cos(q2L)*((6283307137322267*cos(q1L))/9007199254740992 - (4872700232219253*sin(q1L))/9007199254740992))/36893488147419103232 - (76229820211215127867025072518845*cos(q2L))/162259276829213363391578010288128 + sin(q2L)*((4872700232219253*cos(q1L))/9007199254740992 + (6283307137322267*sin(q1L))/9007199254740992)))/36893488147419103232 - sin(q3L)*((76229820211215127867025072518845*sin(q2L))/162259276829213363391578010288128 + cos(q2L)*((4872700232219253*cos(q1L))/9007199254740992 + (6283307137322267*sin(q1L))/9007199254740992) - (7514214926474921*sin(q2L)*((6283307137322267*cos(q1L))/9007199254740992 - (4872700232219253*sin(q1L))/9007199254740992))/36893488147419103232)))/36893488147419103232)))/36893488147419103232000 + (324259171862923063*cos(q6L)*((9007199067919185*sin(q5L)*((666467732349846997487583938718911583194406904318712922873589125*cos(q1L))/113078212145816597093331040047546785012958969400039613319782796882727665664 + (1076049180065244948668759145796765391250102872519935285209856875*cos(q2L))/55213970774324510299478046898216203619608871777363092441300193790394368 - (516845254133432670685844229576986303733782399690601453662320875*sin(q1L))/113078212145816597093331040047546785012958969400039613319782796882727665664 - (81129635049124235038645691064225*cos(q3L)*((56594998190739085871744456992395*cos(q1L))/81129638414606681695789005144064 - (43889380989894851923989405068805*sin(q1L))/81129638414606681695789005144064 + 63594381400292563045725890951477/664613997892457936451903530140172288))/81129638414606681695789005144064 + (2115063383689692319117831580025*sin(q3L)*((56594998190739085871744456992395*cos(q1L))/81129638414606681695789005144064 - (43889380989894851923989405068805*sin(q1L))/81129638414606681695789005144064 + 63594381400292563045725890951477/664613997892457936451903530140172288))/10384593717069655257060992658440192 - (67682029681889335677290557259385*cos(q3L)*((7514214926474921*cos(q2L)*((6283307137322267*cos(q1L))/9007199254740992 - (4872700232219253*sin(q1L))/9007199254740992))/36893488147419103232 - (76229820211215127867025072518845*cos(q2L))/162259276829213363391578010288128 + sin(q2L)*((4872700232219253*cos(q1L))/9007199254740992 + (6283307137322267*sin(q1L))/9007199254740992)))/332306998946228968225951765070086144 + (234819211581865*cos(q3L)*((76229820211215127867025072518845*sin(q2L))/162259276829213363391578010288128 + cos(q2L)*((4872700232219253*cos(q1L))/9007199254740992 + (6283307137322267*sin(q1L))/9007199254740992) - (7514214926474921*sin(q2L)*((6283307137322267*cos(q1L))/9007199254740992 - (4872700232219253*sin(q1L))/9007199254740992))/36893488147419103232))/1152921504606846976 + (1764482024691522628700660907665*sin(q3L)*((7514214926474921*cos(q2L)*((6283307137322267*cos(q1L))/9007199254740992 - (4872700232219253*sin(q1L))/9007199254740992))/36893488147419103232 - (76229820211215127867025072518845*cos(q2L))/162259276829213363391578010288128 + sin(q2L)*((4872700232219253*cos(q1L))/9007199254740992 + (6283307137322267*sin(q1L))/9007199254740992)))/42535295865117307932921825928971026432 + (9007199067919185*sin(q3L)*((76229820211215127867025072518845*sin(q2L))/162259276829213363391578010288128 + cos(q2L)*((4872700232219253*cos(q1L))/9007199254740992 + (6283307137322267*sin(q1L))/9007199254740992) - (7514214926474921*sin(q2L)*((6283307137322267*cos(q1L))/9007199254740992 - (4872700232219253*sin(q1L))/9007199254740992))/36893488147419103232))/9007199254740992 - (106069577339469832923929692356850887620017617375*cos(q2L)*((6283307137322267*cos(q1L))/9007199254740992 - (4872700232219253*sin(q1L))/9007199254740992))/12554203470773361527671578846415332832204710888928069025792 - (14115856197532180673579726082375*sin(q2L)*((4872700232219253*cos(q1L))/9007199254740992 + (6283307137322267*sin(q1L))/9007199254740992))/340282366920938463463374607431768211456 + 748893091562634003789577347105888574211761174637088840996300475/926336713898529563388567880069503262826159877325124512315660672063305037119488))/9007199254740992 - (7514214926474921*sin(q5L)*(((4503599440548691*cos(q4L))/4503599627370496 - (7514214926474921*sin(q4L))/36893488147419103232)*((9007199067919185*sin(q3L)*((56594998190739085871744456992395*cos(q1L))/81129638414606681695789005144064 - (43889380989894851923989405068805*sin(q1L))/81129638414606681695789005144064 + 63594381400292563045725890951477/664613997892457936451903530140172288))/9007199254740992 + cos(q3L)*((76229820211215127867025072518845*sin(q2L))/162259276829213363391578010288128 + 